simulink model "myrobot"  (R2019b)
(part 5 of 7)

-theta2_dot.*(((cos(theta1).*cos(theta2).*sin(theta3).*6.228833385e-1+cos(theta1).*cos(theta3).*sin(theta2).*6.228833385e-1).*(cos(theta1).*cos(theta2).*(4.3e+1./1.0e+2)-cos(theta1).*sin(theta2).*sin(theta3).*1.20975e-1+cos(theta1).*cos(theta2).*cos(theta3).*1.20975e-1))./2.0+((cos(theta2).*sin(theta1).*sin(theta3).*6.228833385e-1+cos(theta3).*sin(theta1).*sin(theta2).*6.228833385e-1).*(cos(theta2).*sin(theta1).*(4.3e+1./1.0e+2)-sin(theta1).*sin(theta2).*sin(theta3).*1.20975e-1+cos(theta2).*cos(theta3).*sin(theta1).*1.20975e-1))./2.0-((cos(theta2).*cos(theta3).*1.20975e-1-sin(theta2).*sin(theta3).*1.20975e-1).*(sin(theta2).*2.2140098+cos(theta2).*sin(theta3).*6.228833385e-1+cos(theta3).*sin(theta2).*6.228833385e-1))./2.0+((cos(theta1).*cos(theta2).*sin(theta3).*1.20975e-1+cos(theta1).*cos(theta3).*sin(theta2).*1.20975e-1).*(cos(theta1).*cos(theta2).*2.2140098-cos(theta1).*sin(theta2).*sin(theta3).*6.228833385e-1+cos(theta1).*cos(theta2).*cos(theta3).*6.228833385e-1))./2.0+(cos(theta1).*(sin(theta1).*(cos(theta1).*(cos(theta1).*sin(theta2).*sin(theta3).*(-2.74946e-3)+cos(theta1).*cos(theta2).*cos(theta3).*2.74946e-3+cos(theta1).*cos(theta2).*sin(theta3).*2.13561e-9+cos(theta1).*cos(theta3).*sin(theta2).*2.13561e-9)+(cos(theta2).*sin(theta1).*sin(theta3)+cos(theta3).*sin(theta1).*sin(theta2)).*(sin(theta1).*(-2.13561e-9)+cos(theta1).*sin(theta2).*sin(theta3).*7.5434e-2-cos(theta1).*cos(theta2).*cos(theta3).*7.5434e-2+cos(theta1).*cos(theta2).*sin(theta3).*2.67415e-8+cos(theta1).*cos(theta3).*sin(theta2).*2.67415e-8)+(cos(theta2).*sin(theta1).*sin(theta3)+cos(theta3).*sin(theta1).*sin(theta2)).*(cos(theta1).*sin(theta2).*sin(theta3).*(-1.0425e-2)+cos(theta1).*cos(theta2).*cos(theta3).*1.0425e-2+cos(theta1).*cos(theta2).*sin(theta3).*2.67415e-8+cos(theta1).*cos(theta3).*sin(theta2).*2.67415e-8)+(sin(theta1).*sin(theta2).*sin(theta3)-cos(theta2).*cos(theta3).*sin(theta1)).*(cos(theta1).*sin(theta2).*sin(theta3).*(-2.67415e-8)+cos(theta1).*cos(theta2).*cos(theta3).*2.67415e-8+cos(theta1).*cos(theta2).*sin(theta3).*7.5434e-2+cos(theta1).*cos(theta3).*sin(theta2).*7.5434e-2)-(sin(theta1).*sin(theta2).*sin(theta3)-cos(theta2).*cos(theta3).*sin(theta1)).*(sin(theta1).*(-2.74946e-3)+cos(theta1).*sin(theta2).*sin(theta3).*2.67415e-8-cos(theta1).*cos(theta2).*cos(theta3).*2.67415e-8+cos(theta1).*cos(theta2).*sin(theta3).*1.0425e-2+cos(theta1).*cos(theta3).*sin(theta2).*1.0425e-2))-cos(theta1).*((sin(theta1).*sin(theta2).*sin(theta3)-cos(theta2).*cos(theta3).*sin(theta1)).*(cos(theta2).*sin(theta1).*sin(theta3).*7.5434e-2+cos(theta3).*sin(theta1).*sin(theta2).*7.5434e-2-sin(theta1).*sin(theta2).*sin(theta3).*2.67415e-8+cos(theta2).*cos(theta3).*sin(theta1).*2.67415e-8)-(sin(theta1).*sin(theta2).*sin(theta3)-cos(theta2).*cos(theta3).*sin(theta1)).*(cos(theta1).*2.74946e-3+cos(theta2).*sin(theta1).*sin(theta3).*1.0425e-2+cos(theta3).*sin(theta1).*sin(theta2).*1.0425e-2+sin(theta1).*sin(theta2).*sin(theta3).*2.67415e-8-cos(theta2).*cos(theta3).*sin(theta1).*2.67415e-8)+(cos(theta2).*sin(theta1).*sin(theta3)+cos(theta3).*sin(theta1).*sin(theta2)).*(cos(theta1).*2.13561e-9+cos(theta2).*sin(theta1).*sin(theta3).*2.67415e-8+cos(theta3).*sin(theta1).*sin(theta2).*2.67415e-8+sin(theta1).*sin(theta2).*sin(theta3).*7.5434e-2-cos(theta2).*cos(theta3).*sin(theta1).*7.5434e-2)+cos(theta1).*(cos(theta2).*sin(theta1).*sin(theta3).*2.13561e-9+cos(theta3).*sin(theta1).*sin(theta2).*2.13561e-9-sin(theta1).*sin(theta2).*sin(theta3).*2.74946e-3+cos(theta2).*cos(theta3).*sin(theta1).*2.74946e-3)+(cos(theta2).*sin(theta1).*sin(theta3)+cos(theta3).*sin(theta1).*sin(theta2)).*(cos(theta2).*sin(theta1).*sin(theta3).*2.67415e-8+cos(theta3).*sin(theta1).*sin(theta2).*2.67415e-8-sin(theta1).*sin(theta2).*sin(theta3).*1.0425e-2+cos(theta2).*cos(theta3).*sin(theta1).*1.0425e-2))))./2.0+((cos(theta2).*sin(theta1).*sin(theta3).*1.20975e-1+cos(theta3).*sin(theta1).*sin(theta2).*1.20975e-1).*(cos(theta2).*sin(theta1).*2.2140098-sin(theta1).*sin(theta2).*sin(theta3).*6.228833385e-1+cos(theta2).*cos(theta3).*sin(theta1).*6.228833385e-1))./2.0-((cos(theta2).*cos(theta3).*6.228833385e-1-sin(theta2).*sin(theta3).*6.228833385e-1).*(sin(theta2).*(4.3e+1./1.0e+2)+cos(theta2).*sin(theta3).*1.20975e-1+cos(theta3).*sin(theta2).*1.20975e-1))./2.0-(sin(theta1).*(sin(theta1).*((cos(theta1).*cos(theta2).*sin(theta3)+cos(theta1).*cos(theta3).*sin(theta2)).*(sin(theta1).*(-2.13561e-9)+cos(theta1).*sin(theta2).*sin(theta3).*7.5434e-2-cos(theta1).*cos(theta2).*cos(theta3).*7.5434e-2+cos(theta1).*cos(theta2).*sin(theta3).*2.67415e-8+cos(theta1).*cos(theta3).*sin(theta2).*2.67415e-8)+(cos(theta1).*cos(theta2).*sin(theta3)+cos(theta1).*cos(theta3).*sin(theta2)).*(cos(theta1).*sin(theta2).*sin(theta3).*(-1.0425e-2)+cos(theta1).*cos(theta2).*cos(theta3).*1.0425e-2+cos(theta1).*cos(theta2).*sin(theta3).*2.67415e-8+cos(theta1).*cos(theta3).*sin(theta2).*2.67415e-8)-sin(theta1).*(cos(theta1).*sin(theta2).*sin(theta3).*(-2.74946e-3)+cos(theta1).*cos(theta2).*cos(theta3).*2.74946e-3+cos(theta1).*cos(theta2).*sin(theta3).*2.13561e-9+cos(theta1).*cos(theta3).*sin(theta2).*2.13561e-9)+(cos(theta1).*sin(theta2).*sin(theta3)-cos(theta1).*cos(theta2).*cos(theta3)).*(cos(theta1).*sin(theta2).*sin(theta3).*(-2.67415e-8)+cos(theta1).*cos(theta2).*cos(theta3).*2.67415e-8+cos(theta1).*cos(theta2).*sin(theta3).*7.5434e-2+cos(theta1).*cos(theta3).*sin(theta2).*7.5434e-2)-(cos(theta1).*sin(theta2).*sin(theta3)-cos(theta1).*cos(theta2).*cos(theta3)).*(sin(theta1).*(-2.74946e-3)+cos(theta1).*sin(theta2).*sin(theta3).*2.67415e-8-cos(theta1).*cos(theta2).*cos(theta3).*2.67415e-8+cos(theta1).*cos(theta2).*sin(theta3).*1.0425e-2+cos(theta1).*cos(theta3).*sin(theta2).*1.0425e-2))-cos(theta1).*((cos(theta1).*cos(theta2).*sin(theta3)+cos(theta1).*cos(theta3).*sin(theta2)).*(cos(theta1).*2.13561e-9+cos(theta2).*sin(theta1).*sin(theta3).*2.67415e-8+cos(theta3).*sin(theta1).*sin(theta2).*2.67415e-8+sin(theta1).*sin(theta2).*sin(theta3).*7.5434e-2-cos(theta2).*cos(theta3).*sin(theta1).*7.5434e-2)+(cos(theta1).*cos(theta2).*sin(theta3)+cos(theta1).*cos(theta3).*sin(theta2)).*(cos(theta2).*sin(theta1).*sin(theta3).*2.67415e-8+cos(theta3).*sin(theta1).*sin(theta2).*2.67415e-8-sin(theta1).*sin(theta2).*sin(theta3).*1.0425e-2+cos(theta2).*cos(theta3).*sin(theta1).*1.0425e-2)-sin(theta1).*(cos(theta2).*sin(theta1).*sin(theta3).*2.13561e-9+cos(theta3).*sin(theta1).*sin(theta2).*2.13561e-9-sin(theta1).*sin(theta2).*sin(theta3).*2.74946e-3+cos(theta2).*cos(theta3).*sin(theta1).*2.74946e-3)+(cos(theta1).*sin(theta2).*sin(theta3)-cos(theta1).*cos(theta2).*cos(theta3)).*(cos(theta2).*sin(theta1).*sin(theta3).*7.5434e-2+cos(theta3).*sin(theta1).*sin(theta2).*7.5434e-2-sin(theta1).*sin(theta2).*sin(theta3).*2.67415e-8+cos(theta2).*cos(theta3).*sin(theta1).*2.67415e-8)-(cos(theta1).*sin(theta2).*sin(theta3)-cos(theta1).*cos(theta2).*cos(theta3)).*(cos(theta1).*2.74946e-3+cos(theta2).*sin(theta1).*sin(theta3).*1.0425e-2+cos(theta3).*sin(theta1).*sin(theta2).*1.0425e-2+sin(theta1).*sin(theta2).*sin(theta3).*2.67415e-8-cos(theta2).*cos(theta3).*sin(theta1).*2.67415e-8))))./2.0)-theta3_dot.*(((cos(theta2).*sin(theta1).*sin(theta3).*1.20975e-1+cos(theta3).*sin(theta1).*sin(theta2).*1.20975e-1).*(sin(theta1).*sin(theta2).*sin(theta3).*6.228833385e-1-cos(theta2).*cos(theta3).*sin(theta1).*6.228833385e-1))./2.0-((sin(theta1).*sin(theta2).*sin(theta3).*1.20975e-1-cos(theta2).*cos(theta3).*sin(theta1).*1.20975e-1).*(cos(theta2).*sin(theta1).*sin(theta3).*6.228833385e-1+cos(theta3).*sin(theta1).*sin(theta2).*6.228833385e-1))./2.0-(cos(theta2).*cos(theta3).*1.20975e-1-sin(theta2).*sin(theta3).*1.20975e-1).*(sin(theta2).*2.2140098+cos(theta2).*sin(theta3).*6.228833385e-1+cos(theta3).*sin(theta2).*6.228833385e-1)+(cos(theta1).*cos(theta2).*sin(theta3).*1.20975e-1+cos(theta1).*cos(theta3).*sin(theta2).*1.20975e-1).*(cos(theta1).*cos(theta2).*2.2140098-cos(theta1).*sin(theta2).*sin(theta3).*6.228833385e-1+cos(theta1).*cos(theta2).*cos(theta3).*6.228833385e-1)+((cos(theta2).*cos(theta3).*1.20975e-1-sin(theta2).*sin(theta3).*1.20975e-1).*(cos(theta2).*sin(theta3).*6.228833385e-1+cos(theta3).*sin(theta2).*6.228833385e-1))./2.0-((cos(theta2).*sin(theta3).*1.20975e-1+cos(theta3).*sin(theta2).*1.20975e-1).*(cos(theta2).*cos(theta3).*6.228833385e-1-sin(theta2).*sin(theta3).*6.228833385e-1))./2.0+(cos(theta1).*(sin(theta1).*(cos(theta1).*(cos(theta1).*sin(theta2).*sin(theta3).*(-2.74946e-3)+cos(theta1).*cos(theta2).*cos(theta3).*2.74946e-3+cos(theta1).*cos(theta2).*sin(theta3).*2.13561e-9+cos(theta1).*cos(theta3).*sin(theta2).*2.13561e-9)+(cos(theta2).*sin(theta1).*sin(theta3)+cos(theta3).*sin(theta1).*sin(theta2)).*(sin(theta1).*(-2.13561e-9)+cos(theta1).*sin(theta2).*sin(theta3).*7.5434e-2-cos(theta1).*cos(theta2).*cos(theta3).*7.5434e-2+cos(theta1).*cos(theta2).*sin(theta3).*2.67415e-8+cos(theta1).*cos(theta3).*sin(theta2).*2.67415e-8)+(cos(theta2).*sin(theta1).*sin(theta3)+cos(theta3).*sin(theta1).*sin(theta2)).*(cos(theta1).*sin(theta2).*sin(theta3).*(-1.0425e-2)+cos(theta1).*cos(theta2).*cos(theta3).*1.0425e-2+cos(theta1).*cos(theta2).*sin(theta3).*2.67415e-8+cos(theta1).*cos(theta3).*sin(theta2).*2.67415e-8)+(sin(theta1).*sin(theta2).*sin(theta3)-cos(theta2).*cos(theta3).*sin(theta1)).*(cos(theta1).*sin(theta2).*sin(theta3).*(-2.67415e-8)+cos(theta1).*cos(theta2).*cos(theta3).*2.67415e-8+cos(theta1).*cos(theta2).*sin(theta3).*7.5434e-2+cos(theta1).*cos(theta3).*sin(theta2).*7.5434e-2)-(sin(theta1).*sin(theta2).*sin(theta3)-cos(theta2).*cos(theta3).*sin(theta1)).*(sin(theta1).*(-2.74946e-3)+cos(theta1).*sin(theta2).*sin(theta3).*2.67415e-8-cos(theta1).*cos(theta2).*cos(theta3).*2.67415e-8+cos(theta1).*cos(theta2).*sin(theta3).*1.0425e-2+cos(theta1).*cos(theta3).*sin(theta2).*1.0425e-2))-cos(theta1).*((sin(theta1).*sin(theta2).*sin(theta3)-cos(theta2).*cos(theta3).*sin(theta1)).*(cos(theta2).*sin(theta1).*sin(theta3).*7.5434e-2+cos(theta3).*sin(theta1).*sin(theta2).*7.5434e-2-sin(theta1).*sin(theta2).*sin(theta3).*2.67415e-8+cos(theta2).*cos(theta3).*sin(theta1).*2.67415e-8)-(sin(theta1).*sin(theta2).*sin(theta3)-cos(theta2).*cos(theta3).*sin(theta1)).*(cos(theta1).*2.74946e-3+cos(theta2).*sin(theta1).*sin(theta3).*1.0425e-2+cos(theta3).*sin(theta1).*sin(theta2).*1.0425e-2+sin(theta1).*sin(theta2).*sin(theta3).*2.67415e-8-cos(theta2).*cos(theta3).*sin(theta1).*2.67415e-8)+(cos(theta2).*sin(theta1).*sin(theta3)+cos(theta3).*sin(theta1).*sin(theta2)).*(cos(theta1).*2.13561e-9+cos(theta2).*sin(theta1).*sin(theta3).*2.67415e-8+cos(theta3).*sin(theta1).*sin(theta2).*2.67415e-8+sin(theta1).*sin(theta2).*sin(theta3).*7.5434e-2-cos(theta2).*cos(theta3).*sin(theta1).*7.5434e-2)+cos(theta1).*(cos(theta2).*sin(theta1).*sin(theta3).*2.13561e-9+cos(theta3).*sin(theta1).*sin(theta2).*2.13561e-9-sin(theta1).*sin(theta2).*sin(theta3).*2.74946e-3+cos(theta2).*cos(theta3).*sin(theta1).*2.74946e-3)+(cos(theta2).*sin(theta1).*sin(theta3)+cos(theta3).*sin(theta1).*sin(theta2)).*(cos(theta2).*sin(theta1).*sin(theta3).*2.67415e-8+cos(theta3).*sin(theta1).*sin(theta2).*2.67415e-8-sin(theta1).*sin(theta2).*sin(theta3).*1.0425e-2+cos(theta2).*cos(theta3).*sin(theta1).*1.0425e-2))))./2.0+(cos(theta2).*sin(theta1).*sin(theta3).*1.20975e-1+cos(theta3).*sin(theta1).*sin(theta2).*1.20975e-1).*(cos(theta2).*sin(theta1).*2.2140098-sin(theta1).*sin(theta2).*sin(theta3).*6.228833385e-1+cos(theta2).*cos(theta3).*sin(theta1).*6.228833385e-1)-(sin(theta1).*(sin(theta1).*((cos(theta1).*cos(theta2).*sin(theta3)+cos(theta1).*cos(theta3).*sin(theta2)).*(sin(theta1).*(-2.13561e-9)+cos(theta1).*sin(theta2).*sin(theta3).*7.5434e-2-cos(theta1).*cos(theta2).*cos(theta3).*7.5434e-2+cos(theta1).*cos(theta2).*sin(theta3).*2.67415e-8+cos(theta1).*cos(theta3).*sin(theta2).*2.67415e-8)+(cos(theta1).*cos(theta2).*sin(theta3)+cos(theta1).*cos(theta3).*sin(theta2)).*(cos(theta1).*sin(theta2).*sin(theta3).*(-1.0425e-2)+cos(theta1).*cos(theta2).*cos(theta3).*1.0425e-2+cos(theta1).*cos(theta2).*sin(theta3).*2.67415e-8+cos(theta1).*cos(theta3).*sin(theta2).*2.67415e-8)-sin(theta1).*(cos(theta1).*sin(theta2).*sin(theta3).*(-2.74946e-3)+cos(theta1).*cos(theta2).*cos(theta3).*2.74946e-3+cos(theta1).*cos(theta2).*sin(theta3).*2.13561e-9+cos(theta1).*cos(theta3).*sin(theta2).*2.13561e-9)+(cos(theta1).*sin(theta2).*sin(theta3)-cos(theta1).*cos(theta2).*cos(theta3)).*(cos(theta1).*sin(theta2).*sin(theta3).*(-2.67415e-8)+cos(theta1).*cos(theta2).*cos(theta3).*2.67415e-8+cos(theta1).*cos(theta2).*sin(theta3).*7.5434e-2+cos(theta1).*cos(theta3).*sin(theta2).*7.5434e-2)-(cos(theta1).*sin(theta2).*sin(theta3)-cos(theta1).*cos(theta2).*cos(theta3)).*(sin(theta1).*(-2.74946e-3)+cos(theta1).*sin(theta2).*sin(theta3).*2.67415e-8-cos(theta1).*cos(theta2).*cos(theta3).*2.67415e-8+cos(theta1).*cos(theta2).*sin(theta3).*1.0425e-2+cos(theta1).*cos(theta3).*sin(theta2).*1.0425e-2))-cos(theta1).*((cos(theta1).*cos(theta2).*sin(theta3)+cos(theta1).*cos(theta3).*sin(theta2)).*(cos(theta1).*2.13561e-9+cos(theta2).*sin(theta1).*sin(theta3).*2.67415e-8+cos(theta3).*sin(theta1).*sin(theta2).*2.67415e-8+sin(theta1).*sin(theta2).*sin(theta3).*7.5434e-2-cos(theta2).*cos(theta3).*sin(theta1).*7.5434e-2)+(cos(theta1).*cos(theta2).*sin(theta3)+cos(theta1).*cos(theta3).*sin(theta2)).*(cos(theta2).*sin(theta1).*sin(theta3).*2.67415e-8+cos(theta3).*sin(theta1).*sin(theta2).*2.67415e-8-sin(theta1).*sin(theta2).*sin(theta3).*1.0425e-2+cos(theta2).*cos(theta3).*sin(theta1).*1.0425e-2)-sin(theta1).*(cos(theta2).*sin(theta1).*sin(theta3).*2.13561e-9+cos(theta3).*sin(theta1).*sin(theta2).*2.13561e-9-sin(theta1).*sin(theta2).*sin(theta3).*2.74946e-3+cos(theta2).*cos(theta3).*sin(theta1).*2.74946e-3)+(cos(theta1).*sin(theta2).*sin(theta3)-cos(theta1).*cos(theta2).*cos(theta3)).*(cos(theta2).*sin(theta1).*sin(theta3).*7.5434e-2+cos(theta3).*sin(theta1).*sin(theta2).*7.5434e-2-sin(theta1).*sin(theta2).*sin(theta3).*2.67415e-8+cos(theta2).*cos(theta3).*sin(theta1).*2.67415e-8)-(cos(theta1).*sin(theta2).*sin(theta3)-cos(theta1).*cos(theta2).*cos(theta3)).*(cos(theta1).*2.74946e-3+cos(theta2).*sin(theta1).*sin(theta3).*1.0425e-2+cos(theta3).*sin(theta1).*sin(theta2).*1.0425e-2+sin(theta1).*sin(theta2).*sin(theta3).*2.67415e-8-cos(theta2).*cos(theta3).*sin(theta1).*2.67415e-8))))./2.0-((cos(theta1).*sin(theta2).*sin(theta3).*1.20975e-1-cos(theta1).*cos(theta2).*cos(theta3).*1.20975e-1).*(cos(theta1).*cos(theta2).*sin(theta3).*6.228833385e-1+cos(theta1).*cos(theta3).*sin(theta2).*6.228833385e-1))./2.0+((cos(theta1).*cos(theta2).*sin(theta3).*1.20975e-1+cos(theta1).*cos(theta3).*sin(theta2).*1.20975e-1).*(cos(theta1).*sin(theta2).*sin(theta3).*6.228833385e-1-cos(theta1).*cos(theta2).*cos(theta3).*6.228833385e-1))./2.0)-theta1_dot.*((cos(theta1).*(cos(theta1).*(cos(theta1).*(sin(theta1).*(-7.44749e-2)+cos(theta1).*sin(theta2).*sin(theta3).*2.13561e-9-cos(theta1).*cos(theta2).*cos(theta3).*2.13561e-9+cos(theta1).*cos(theta2).*sin(theta3).*2.74946e-3+cos(theta1).*cos(theta3).*sin(theta2).*2.74946e-3)+(sin(theta1).*sin(theta2).*sin(theta3)-cos(theta2).*cos(theta3).*sin(theta1)).*(sin(theta1).*(-2.13561e-9)+cos(theta1).*sin(theta2).*sin(theta3).*7.5434e-2-cos(theta1).*cos(theta2).*cos(theta3).*7.5434e-2+cos(theta1).*cos(theta2).*sin(theta3).*2.67415e-8+cos(theta1).*cos(theta3).*sin(theta2).*2.67415e-8)+(cos(theta2).*sin(theta1).*sin(theta3)+cos(theta3).*sin(theta1).*sin(theta2)).*(sin(theta1).*(-2.74946e-3)+cos(theta1).*sin(theta2).*sin(theta3).*2.67415e-8-cos(theta1).*cos(theta2).*cos(theta3).*2.67415e-8+cos(theta1).*cos(theta2).*sin(theta3).*1.0425e-2+cos(theta1).*cos(theta3).*sin(theta2).*1.0425e-2))+sin(theta1).*((cos(theta2).*sin(theta1).*sin(theta3)+cos(theta3).*sin(theta1).*sin(theta2)).*(cos(theta1).*2.74946e-3+cos(theta2).*sin(theta1).*sin(theta3).*1.0425e-2+cos(theta3).*sin(theta1).*sin(theta2).*1.0425e-2+sin(theta1).*sin(theta2).*sin(theta3).*2.67415e-8-cos(theta2).*cos(theta3).*sin(theta1).*2.67415e-8)+cos(theta1).*(cos(theta1).*7.44749e-2+cos(theta2).*sin(theta1).*sin(theta3).*2.74946e-3+cos(theta3).*sin(theta1).*sin(theta2).*2.74946e-3+sin(theta1).*sin(theta2).*sin(theta3).*2.13561e-9-cos(theta2).*cos(theta3).*sin(theta1).*2.13561e-9)+(sin(theta1).*sin(theta2).*sin(theta3)-cos(theta2).*cos(theta3).*sin(theta1)).*(cos(theta1).*2.13561e-9+cos(theta2).*sin(theta1).*sin(theta3).*2.67415e-8+cos(theta3).*sin(theta1).*sin(theta2).*2.67415e-8+sin(theta1).*sin(theta2).*sin(theta3).*7.5434e-2-cos(theta2).*cos(theta3).*sin(theta1).*7.5434e-2))-cos(theta1).*(cos(theta1).*(sin(theta1).*(-7.44749e-2)+cos(theta1).*sin(theta2).*sin(theta3).*2.13561e-9-cos(theta1).*cos(theta2).*cos(theta3).*2.13561e-9+cos(theta1).*cos(theta2).*sin(theta3).*2.74946e-3+cos(theta1).*cos(theta3).*sin(theta2).*2.74946e-3)+(sin(theta1).*sin(theta2).*sin(theta3)-cos(theta2).*cos(theta3).*sin(theta1)).*(sin(theta1).*(-2.13561e-9)+cos(theta1).*sin(theta2).*sin(theta3).*7.5434e-2-cos(theta1).*cos(theta2).*cos(theta3).*7.5434e-2+cos(theta1).*cos(theta2).*sin(theta3).*2.67415e-8+cos(theta1).*cos(theta3).*sin(theta2).*2.67415e-8)-sin(theta1).*(cos(theta1).*7.44749e-2+cos(theta2).*sin(theta1).*sin(theta3).*2.74946e-3+cos(theta3).*sin(theta1).*sin(theta2).*2.74946e-3+sin(theta1).*sin(theta2).*sin(theta3).*2.13561e-9-cos(theta2).*cos(theta3).*sin(theta1).*2.13561e-9)+(cos(theta1).*sin(theta2).*sin(theta3)-cos(theta1).*cos(theta2).*cos(theta3)).*(cos(theta1).*2.13561e-9+cos(theta2).*sin(theta1).*sin(theta3).*2.67415e-8+cos(theta3).*sin(theta1).*sin(theta2).*2.67415e-8+sin(theta1).*sin(theta2).*sin(theta3).*7.5434e-2-cos(theta2).*cos(theta3).*sin(theta1).*7.5434e-2)+(cos(theta2).*sin(theta1).*sin(theta3)+cos(theta3).*sin(theta1).*sin(theta2)).*(sin(theta1).*(-2.74946e-3)+cos(theta1).*sin(theta2).*sin(theta3).*2.67415e-8-cos(theta1).*cos(theta2).*cos(theta3).*2.67415e-8+cos(theta1).*cos(theta2).*sin(theta3).*1.0425e-2+cos(theta1).*cos(theta3).*sin(theta2).*1.0425e-2)+(cos(theta1).*cos(theta2).*sin(theta3)+cos(theta1).*cos(theta3).*sin(theta2)).*(cos(theta1).*2.74946e-3+cos(theta2).*sin(theta1).*sin(theta3).*1.0425e-2+cos(theta3).*sin(theta1).*sin(theta2).*1.0425e-2+sin(theta1).*sin(theta2).*sin(theta3).*2.67415e-8-cos(theta2).*cos(theta3).*sin(theta1).*2.67415e-8))-sin(theta1).*((cos(theta2).*sin(theta1).*sin(theta3)+cos(theta3).*sin(theta1).*sin(theta2)).*(cos(theta1).*2.74946e-3+cos(theta2).*sin(theta1).*sin(theta3).*1.0425e-2+cos(theta3).*sin(theta1).*sin(theta2).*1.0425e-2+sin(theta1).*sin(theta2).*sin(theta3).*2.67415e-8-cos(theta2).*cos(theta3).*sin(theta1).*2.67415e-8)+sin(theta1).*(sin(theta1).*(-7.44749e-2)+cos(theta1).*sin(theta2).*sin(theta3).*2.13561e-9-cos(theta1).*cos(theta2).*cos(theta3).*2.13561e-9+cos(theta1).*cos(theta2).*sin(theta3).*2.74946e-3+cos(theta1).*cos(theta3).*sin(theta2).*2.74946e-3)-(cos(theta1).*sin(theta2).*sin(theta3)-cos(theta1).*cos(theta2).*cos(theta3)).*(sin(theta1).*(-2.13561e-9)+cos(theta1).*sin(theta2).*sin(theta3).*7.5434e-2-cos(theta1).*cos(theta2).*cos(theta3).*7.5434e-2+cos(theta1).*cos(theta2).*sin(theta3).*2.67415e-8+cos(theta1).*cos(theta3).*sin(theta2).*2.67415e-8)+cos(theta1).*(cos(theta1).*7.44749e-2+cos(theta2).*sin(theta1).*sin(theta3).*2.74946e-3+cos(theta3).*sin(theta1).*sin(theta2).*2.74946e-3+sin(theta1).*sin(theta2).*sin(theta3).*2.13561e-9-cos(theta2).*cos(theta3).*sin(theta1).*2.13561e-9)+(sin(theta1).*sin(theta2).*sin(theta3)-cos(theta2).*cos(theta3).*sin(theta1)).*(cos(theta1).*2.13561e-9+cos(theta2).*sin(theta1).*sin(theta3).*2.67415e-8+cos(theta3).*sin(theta1).*sin(theta2).*2.67415e-8+sin(theta1).*sin(theta2).*sin(theta3).*7.5434e-2-cos(theta2).*cos(theta3).*sin(theta1).*7.5434e-2)-(cos(theta1).*cos(theta2).*sin(theta3)+cos(theta1).*cos(theta3).*sin(theta2)).*(sin(theta1).*(-2.74946e-3)+cos(theta1).*sin(theta2).*sin(theta3).*2.67415e-8-cos(theta1).*cos(theta2).*cos(theta3).*2.67415e-8+cos(theta1).*cos(theta2).*sin(theta3).*1.0425e-2+cos(theta1).*cos(theta3).*sin(theta2).*1.0425e-2))))./2.0+((cos(theta1).*cos(theta2).*sin(theta3).*1.20975e-1+cos(theta1).*cos(theta3).*sin(theta2).*1.20975e-1).*(cos(theta1).*2.272809781200003e-2+sin(theta1).*sin(theta2).*2.2140098+cos(theta2).*sin(theta1).*sin(theta3).*6.228833385e-1+cos(theta3).*sin(theta1).*sin(theta2).*6.228833385e-1))./2.0-((cos(theta2).*sin(theta1).*sin(theta3).*1.20975e-1+cos(theta3).*sin(theta1).*sin(theta2).*1.20975e-1).*(sin(theta1).*(-2.272809781200003e-2)+cos(theta1).*sin(theta2).*2.2140098+cos(theta1).*cos(theta2).*sin(theta3).*6.228833385e-1+cos(theta1).*cos(theta3).*sin(theta2).*6.228833385e-1))./2.0-((cos(theta1).*cos(theta2).*sin(theta3).*6.228833385e-1+cos(theta1).*cos(theta3).*sin(theta2).*6.228833385e-1).*(cos(theta1).*4.414200000000005e-3+sin(theta1).*sin(theta2).*(4.3e+1./1.0e+2)+cos(theta2).*sin(theta1).*sin(theta3).*1.20975e-1+cos(theta3).*sin(theta1).*sin(theta2).*1.20975e-1))./2.0+((cos(theta2).*sin(theta1).*sin(theta3).*6.228833385e-1+cos(theta3).*sin(theta1).*sin(theta2).*6.228833385e-1).*(sin(theta1).*(-4.414200000000005e-3)+cos(theta1).*sin(theta2).*(4.3e+1./1.0e+2)+cos(theta1).*cos(theta2).*sin(theta3).*1.20975e-1+cos(theta1).*cos(theta3).*sin(theta2).*1.20975e-1))./2.0+(sin(theta1).*(-sin(theta1).*(cos(theta2).*cos(theta3).*(-2.13561e-9)+cos(theta2).*sin(theta3).*2.74946e-3+cos(theta3).*sin(theta2).*2.74946e-3+sin(theta2).*sin(theta3).*2.13561e-9)-(cos(theta1).*cos(theta2).*sin(theta3)+cos(theta1).*cos(theta3).*sin(theta2)).*(cos(theta2).*cos(theta3).*2.67415e-8+cos(theta2).*sin(theta3).*7.5434e-2+cos(theta3).*sin(theta2).*7.5434e-2-sin(theta2).*sin(theta3).*2.67415e-8)+(cos(theta1).*sin(theta2).*sin(theta3)-cos(theta1).*cos(theta2).*cos(theta3)).*(cos(theta2).*cos(theta3).*(-7.5434e-2)+cos(theta2).*sin(theta3).*2.67415e-8+cos(theta3).*sin(theta2).*2.67415e-8+sin(theta2).*sin(theta3).*7.5434e-2)+(cos(theta1).*cos(theta2).*sin(theta3)+cos(theta1).*cos(theta3).*sin(theta2)).*(cos(theta2).*cos(theta3).*(-2.67415e-8)+cos(theta2).*sin(theta3).*1.0425e-2+cos(theta3).*sin(theta2).*1.0425e-2+sin(theta2).*sin(theta3).*2.67415e-8)+(cos(theta1).*sin(theta2).*sin(theta3)-cos(theta1).*cos(theta2).*cos(theta3)).*(cos(theta2).*cos(theta3).*1.0425e-2+cos(theta2).*sin(theta3).*2.67415e-8+cos(theta3).*sin(theta2).*2.67415e-8-sin(theta2).*sin(theta3).*1.0425e-2)))./2.0-(sin(theta1).*(sin(theta1).*(cos(theta1).*(sin(theta1).*(-7.44749e-2)+cos(theta1).*sin(theta2).*sin(theta3).*2.13561e-9-cos(theta1).*cos(theta2).*cos(theta3).*2.13561e-9+cos(theta1).*cos(theta2).*sin(theta3).*2.74946e-3+cos(theta1).*cos(theta3).*sin(theta2).*2.74946e-3)+(sin(theta1).*sin(theta2).*sin(theta3)-cos(theta2).*cos(theta3).*sin(theta1)).*(sin(theta1).*(-2.13561e-9)+cos(theta1).*sin(theta2).*sin(theta3).*7.5434e-2-cos(theta1).*cos(theta2).*cos(theta3).*7.5434e-2+cos(theta1).*cos(theta2).*sin(theta3).*2.67415e-8+cos(theta1).*cos(theta3).*sin(theta2).*2.67415e-8)+(cos(theta2).*sin(theta1).*sin(theta3)+cos(theta3).*sin(theta1).*sin(theta2)).*(sin(theta1).*(-2.74946e-3)+cos(theta1).*sin(theta2).*sin(theta3).*2.67415e-8-cos(theta1).*cos(theta2).*cos(theta3).*2.67415e-8+cos(theta1).*cos(theta2).*sin(theta3).*1.0425e-2+cos(theta1).*cos(theta3).*sin(theta2).*1.0425e-2))-cos(theta1).*((cos(theta2).*sin(theta1).*sin(theta3)+cos(theta3).*sin(theta1).*sin(theta2)).*(cos(theta1).*2.74946e-3+cos(theta2).*sin(theta1).*sin(theta3).*1.0425e-2+cos(theta3).*sin(theta1).*sin(theta2).*1.0425e-2+sin(theta1).*sin(theta2).*sin(theta3).*2.67415e-8-cos(theta2).*cos(theta3).*sin(theta1).*2.67415e-8)+cos(theta1).*(cos(theta1).*7.44749e-2+cos(theta2).*sin(theta1).*sin(theta3).*2.74946e-3+cos(theta3).*sin(theta1).*sin(theta2).*2.74946e-3+sin(theta1).*sin(theta2).*sin(theta3).*2.13561e-9-cos(theta2).*cos(theta3).*sin(theta1).*2.13561e-9)+(sin(theta1).*sin(theta2).*sin(theta3)-cos(theta2).*cos(theta3).*sin(theta1)).*(cos(theta1).*2.13561e-9+cos(theta2).*sin(theta1).*sin(theta3).*2.67415e-8+cos(theta3).*sin(theta1).*sin(theta2).*2.67415e-8+sin(theta1).*sin(theta2).*sin(theta3).*7.5434e-2-cos(theta2).*cos(theta3).*sin(theta1).*7.5434e-2))))./2.0-(cos(theta1).*(cos(theta1).*(cos(theta2).*cos(theta3).*(-2.13561e-9)+cos(theta2).*sin(theta3).*2.74946e-3+cos(theta3).*sin(theta2).*2.74946e-3+sin(theta2).*sin(theta3).*2.13561e-9)+(cos(theta2).*sin(theta1).*sin(theta3)+cos(theta3).*sin(theta1).*sin(theta2)).*(cos(theta2).*cos(theta3).*(-2.67415e-8)+cos(theta2).*sin(theta3).*1.0425e-2+cos(theta3).*sin(theta2).*1.0425e-2+sin(theta2).*sin(theta3).*2.67415e-8)+(sin(theta1).*sin(theta2).*sin(theta3)-cos(theta2).*cos(theta3).*sin(theta1)).*(cos(theta2).*cos(theta3).*1.0425e-2+cos(theta2).*sin(theta3).*2.67415e-8+cos(theta3).*sin(theta2).*2.67415e-8-sin(theta2).*sin(theta3).*1.0425e-2)-(cos(theta2).*sin(theta1).*sin(theta3)+cos(theta3).*sin(theta1).*sin(theta2)).*(cos(theta2).*cos(theta3).*2.67415e-8+cos(theta2).*sin(theta3).*7.5434e-2+cos(theta3).*sin(theta2).*7.5434e-2-sin(theta2).*sin(theta3).*2.67415e-8)+(sin(theta1).*sin(theta2).*sin(theta3)-cos(theta2).*cos(theta3).*sin(theta1)).*(cos(theta2).*cos(theta3).*(-7.5434e-2)+cos(theta2).*sin(theta3).*2.67415e-8+cos(theta3).*sin(theta2).*2.67415e-8+sin(theta2).*sin(theta3).*7.5434e-2)))./2.0-(sin(theta1).*sin(theta2).*sin(theta3).*1.20975e-1-cos(theta2).*cos(theta3).*sin(theta1).*1.20975e-1).*(cos(theta1).*cos(theta2).*2.2140098-cos(theta1).*sin(theta2).*sin(theta3).*6.228833385e-1+cos(theta1).*cos(theta2).*cos(theta3).*6.228833385e-1)-(cos(theta1).*((cos(theta2).*sin(theta3)+cos(theta3).*sin(theta2)).*(cos(theta2).*sin(theta1).*sin(theta3).*7.5434e-2+cos(theta3).*sin(theta1).*sin(theta2).*7.5434e-2-sin(theta1).*sin(theta2).*sin(theta3).*2.67415e-8+cos(theta2).*cos(theta3).*sin(theta1).*2.67415e-8)-(cos(theta2).*sin(theta3)+cos(theta3).*sin(theta2)).*(cos(theta1).*2.74946e-3+cos(theta2).*sin(theta1).*sin(theta3).*1.0425e-2+cos(theta3).*sin(theta1).*sin(theta2).*1.0425e-2+sin(theta1).*sin(theta2).*sin(theta3).*2.67415e-8-cos(theta2).*cos(theta3).*sin(theta1).*2.67415e-8)+(cos(theta2).*cos(theta3)-sin(theta2).*sin(theta3)).*(cos(theta1).*2.13561e-9+cos(theta2).*sin(theta1).*sin(theta3).*2.67415e-8+cos(theta3).*sin(theta1).*sin(theta2).*2.67415e-8+sin(theta1).*sin(theta2).*sin(theta3).*7.5434e-2-cos(theta2).*cos(theta3).*sin(theta1).*7.5434e-2)+(cos(theta2).*cos(theta3)-sin(theta2).*sin(theta3)).*(cos(theta2).*sin(theta1).*sin(theta3).*2.67415e-8+cos(theta3).*sin(theta1).*sin(theta2).*2.67415e-8-sin(theta1).*sin(theta2).*sin(theta3).*1.0425e-2+cos(theta2).*cos(theta3).*sin(theta1).*1.0425e-2)))./2.0+(cos(theta1).*sin(theta2).*sin(theta3).*1.20975e-1-cos(theta1).*cos(theta2).*cos(theta3).*1.20975e-1).*(cos(theta2).*sin(theta1).*2.2140098-sin(theta1).*sin(theta2).*sin(theta3).*6.228833385e-1+cos(theta2).*cos(theta3).*sin(theta1).*6.228833385e-1)-(sin(theta1).*(sin(theta1).*(-sin(theta1).*(cos(theta1).*7.44749e-2+cos(theta2).*sin(theta1).*sin(theta3).*2.74946e-3+cos(theta3).*sin(theta1).*sin(theta2).*2.74946e-3+sin(theta1).*sin(theta2).*sin(theta3).*2.13561e-9-cos(theta2).*cos(theta3).*sin(theta1).*2.13561e-9)+(cos(theta1).*sin(theta2).*sin(theta3)-cos(theta1).*cos(theta2).*cos(theta3)).*(cos(theta1).*2.13561e-9+cos(theta2).*sin(theta1).*sin(theta3).*2.67415e-8+cos(theta3).*sin(theta1).*sin(theta2).*2.67415e-8+sin(theta1).*sin(theta2).*sin(theta3).*7.5434e-2-cos(theta2).*cos(theta3).*sin(theta1).*7.5434e-2)+(cos(theta1).*cos(theta2).*sin(theta3)+cos(theta1).*cos(theta3).*sin(theta2)).*(cos(theta1).*2.74946e-3+cos(theta2).*sin(theta1).*sin(theta3).*1.0425e-2+cos(theta3).*sin(theta1).*sin(theta2).*1.0425e-2+sin(theta1).*sin(theta2).*sin(theta3).*2.67415e-8-cos(theta2).*cos(theta3).*sin(theta1).*2.67415e-8))+cos(theta1).*(-sin(theta1).*(sin(theta1).*(-7.44749e-2)+cos(theta1).*sin(theta2).*sin(theta3).*2.13561e-9-cos(theta1).*cos(theta2).*cos(theta3).*2.13561e-9+cos(theta1).*cos(theta2).*sin(theta3).*2.74946e-3+cos(theta1).*cos(theta3).*sin(theta2).*2.74946e-3)+(cos(theta1).*sin(theta2).*sin(theta3)-cos(theta1).*cos(theta2).*cos(theta3)).*(sin(theta1).*(-2.13561e-9)+cos(theta1).*sin(theta2).*sin(theta3).*7.5434e-2-cos(theta1).*cos(theta2).*cos(theta3).*7.5434e-2+cos(theta1).*cos(theta2).*sin(theta3).*2.67415e-8+cos(theta1).*cos(theta3).*sin(theta2).*2.67415e-8)+(cos(theta1).*cos(theta2).*sin(theta3)+cos(theta1).*cos(theta3).*sin(theta2)).*(sin(theta1).*(-2.74946e-3)+cos(theta1).*sin(theta2).*sin(theta3).*2.67415e-8-cos(theta1).*cos(theta2).*cos(theta3).*2.67415e-8+cos(theta1).*cos(theta2).*sin(theta3).*1.0425e-2+cos(theta1).*cos(theta3).*sin(theta2).*1.0425e-2))+cos(theta1).*((cos(theta2).*sin(theta1).*sin(theta3)+cos(theta3).*sin(theta1).*sin(theta2)).*(cos(theta1).*2.74946e-3+cos(theta2).*sin(theta1).*sin(theta3).*1.0425e-2+cos(theta3).*sin(theta1).*sin(theta2).*1.0425e-2+sin(theta1).*sin(theta2).*sin(theta3).*2.67415e-8-cos(theta2).*cos(theta3).*sin(theta1).*2.67415e-8)+sin(theta1).*(sin(theta1).*(-7.44749e-2)+cos(theta1).*sin(theta2).*sin(theta3).*2.13561e-9-cos(theta1).*cos(theta2).*cos(theta3).*2.13561e-9+cos(theta1).*cos(theta2).*sin(theta3).*2.74946e-3+cos(theta1).*cos(theta3).*sin(theta2).*2.74946e-3)-(cos(theta1).*sin(theta2).*sin(theta3)-cos(theta1).*cos(theta2).*cos(theta3)).*(sin(theta1).*(-2.13561e-9)+cos(theta1).*sin(theta2).*sin(theta3).*7.5434e-2-cos(theta1).*cos(theta2).*cos(theta3).*7.5434e-2+cos(theta1).*cos(theta2).*sin(theta3).*2.67415e-8+cos(theta1).*cos(theta3).*sin(theta2).*2.67415e-8)+cos(theta1).*(cos(theta1).*7.44749e-2+cos(theta2).*sin(theta1).*sin(theta3).*2.74946e-3+cos(theta3).*sin(theta1).*sin(theta2).*2.74946e-3+sin(theta1).*sin(theta2).*sin(theta3).*2.13561e-9-cos(theta2).*cos(theta3).*sin(theta1).*2.13561e-9)+(sin(theta1).*sin(theta2).*sin(theta3)-cos(theta2).*cos(theta3).*sin(theta1)).*(cos(theta1).*2.13561e-9+cos(theta2).*sin(theta1).*sin(theta3).*2.67415e-8+cos(theta3).*sin(theta1).*sin(theta2).*2.67415e-8+sin(theta1).*sin(theta2).*sin(theta3).*7.5434e-2-cos(theta2).*cos(theta3).*sin(theta1).*7.5434e-2)-(cos(theta1).*cos(theta2).*sin(theta3)+cos(theta1).*cos(theta3).*sin(theta2)).*(sin(theta1).*(-2.74946e-3)+cos(theta1).*sin(theta2).*sin(theta3).*2.67415e-8-cos(theta1).*cos(theta2).*cos(theta3).*2.67415e-8+cos(theta1).*cos(theta2).*sin(theta3).*1.0425e-2+cos(theta1).*cos(theta3).*sin(theta2).*1.0425e-2))-sin(theta1).*(cos(theta1).*(sin(theta1).*(-7.44749e-2)+cos(theta1).*sin(theta2).*sin(theta3).*2.13561e-9-cos(theta1).*cos(theta2).*cos(theta3).*2.13561e-9+cos(theta1).*cos(theta2).*sin(theta3).*2.74946e-3+cos(theta1).*cos(theta3).*sin(theta2).*2.74946e-3)+(sin(theta1).*sin(theta2).*sin(theta3)-cos(theta2).*cos(theta3).*sin(theta1)).*(sin(theta1).*(-2.13561e-9)+cos(theta1).*sin(theta2).*sin(theta3).*7.5434e-2-cos(theta1).*cos(theta2).*cos(theta3).*7.5434e-2+cos(theta1).*cos(theta2).*sin(theta3).*2.67415e-8+cos(theta1).*cos(theta3).*sin(theta2).*2.67415e-8)-sin(theta1).*(cos(theta1).*7.44749e-2+cos(theta2).*sin(theta1).*sin(theta3).*2.74946e-3+cos(theta3).*sin(theta1).*sin(theta2).*2.74946e-3+sin(theta1).*sin(theta2).*sin(theta3).*2.13561e-9-cos(theta2).*cos(theta3).*sin(theta1).*2.13561e-9)+(cos(theta1).*sin(theta2).*sin(theta3)-cos(theta1).*cos(theta2).*cos(theta3)).*(cos(theta1).*2.13561e-9+cos(theta2).*sin(theta1).*sin(theta3).*2.67415e-8+cos(theta3).*sin(theta1).*sin(theta2).*2.67415e-8+sin(theta1).*sin(theta2).*sin(theta3).*7.5434e-2-cos(theta2).*cos(theta3).*sin(theta1).*7.5434e-2)+(cos(theta2).*sin(theta1).*sin(theta3)+cos(theta3).*sin(theta1).*sin(theta2)).*(sin(theta1).*(-2.74946e-3)+cos(theta1).*sin(theta2).*sin(theta3).*2.67415e-8-cos(theta1).*cos(theta2).*cos(theta3).*2.67415e-8+cos(theta1).*cos(theta2).*sin(theta3).*1.0425e-2+cos(theta1).*cos(theta3).*sin(theta2).*1.0425e-2)+(cos(theta1).*cos(theta2).*sin(theta3)+cos(theta1).*cos(theta3).*sin(theta2)).*(cos(theta1).*2.74946e-3+cos(theta2).*sin(theta1).*sin(theta3).*1.0425e-2+cos(theta3).*sin(theta1).*sin(theta2).*1.0425e-2+sin(theta1).*sin(theta2).*sin(theta3).*2.67415e-8-cos(theta2).*cos(theta3).*sin(theta1).*2.67415e-8))))./2.0+(sin(theta1).*(-(cos(theta2).*sin(theta3)+cos(theta3).*sin(theta2)).*(sin(theta1).*(-2.74946e-3)+cos(theta1).*sin(theta2).*sin(theta3).*2.67415e-8-cos(theta1).*cos(theta2).*cos(theta3).*2.67415e-8+cos(theta1).*cos(theta2).*sin(theta3).*1.0425e-2+cos(theta1).*cos(theta3).*sin(theta2).*1.0425e-2)+(cos(theta2).*cos(theta3)-sin(theta2).*sin(theta3)).*(sin(theta1).*(-2.13561e-9)+cos(theta1).*sin(theta2).*sin(theta3).*7.5434e-2-cos(theta1).*cos(theta2).*cos(theta3).*7.5434e-2+cos(theta1).*cos(theta2).*sin(theta3).*2.67415e-8+cos(theta1).*cos(theta3).*sin(theta2).*2.67415e-8)+(cos(theta2).*cos(theta3)-sin(theta2).*sin(theta3)).*(cos(theta1).*sin(theta2).*sin(theta3).*(-1.0425e-2)+cos(theta1).*cos(theta2).*cos(theta3).*1.0425e-2+cos(theta1).*cos(theta2).*sin(theta3).*2.67415e-8+cos(theta1).*cos(theta3).*sin(theta2).*2.67415e-8)+(cos(theta2).*sin(theta3)+cos(theta3).*sin(theta2)).*(cos(theta1).*sin(theta2).*sin(theta3).*(-2.67415e-8)+cos(theta1).*cos(theta2).*cos(theta3).*2.67415e-8+cos(theta1).*cos(theta2).*sin(theta3).*7.5434e-2+cos(theta1).*cos(theta3).*sin(theta2).*7.5434e-2)))./2.0+(cos(theta1).*(cos(theta1).*(-sin(theta1).*(cos(theta1).*7.44749e-2+cos(theta2).*sin(theta1).*sin(theta3).*2.74946e-3+cos(theta3).*sin(theta1).*sin(theta2).*2.74946e-3+sin(theta1).*sin(theta2).*sin(theta3).*2.13561e-9-cos(theta2).*cos(theta3).*sin(theta1).*2.13561e-9)+(cos(theta1).*sin(theta2).*sin(theta3)-cos(theta1).*cos(theta2).*cos(theta3)).*(cos(theta1).*2.13561e-9+cos(theta2).*sin(theta1).*sin(theta3).*2.67415e-8+cos(theta3).*sin(theta1).*sin(theta2).*2.67415e-8+sin(theta1).*sin(theta2).*sin(theta3).*7.5434e-2-cos(theta2).*cos(theta3).*sin(theta1).*7.5434e-2)+(cos(theta1).*cos(theta2).*sin(theta3)+cos(theta1).*cos(theta3).*sin(theta2)).*(cos(theta1).*2.74946e-3+cos(theta2).*sin(theta1).*sin(theta3).*1.0425e-2+cos(theta3).*sin(theta1).*sin(theta2).*1.0425e-2+sin(theta1).*sin(theta2).*sin(theta3).*2.67415e-8-cos(theta2).*cos(theta3).*sin(theta1).*2.67415e-8))-sin(theta1).*(-sin(theta1).*(sin(theta1).*(-7.44749e-2)+cos(theta1).*sin(theta2).*sin(theta3).*2.13561e-9-cos(theta1).*cos(theta2).*cos(theta3).*2.13561e-9+cos(theta1).*cos(theta2).*sin(theta3).*2.74946e-3+cos(theta1).*cos(theta3).*sin(theta2).*2.74946e-3)+(cos(theta1).*sin(theta2).*sin(theta3)-cos(theta1).*cos(theta2).*cos(theta3)).*(sin(theta1).*(-2.13561e-9)+cos(theta1).*sin(theta2).*sin(theta3).*7.5434e-2-cos(theta1).*cos(theta2).*cos(theta3).*7.5434e-2+cos(theta1).*cos(theta2).*sin(theta3).*2.67415e-8+cos(theta1).*cos(theta3).*sin(theta2).*2.67415e-8)+(cos(theta1).*cos(theta2).*sin(theta3)+cos(theta1).*cos(theta3).*sin(theta2)).*(sin(theta1).*(-2.74946e-3)+cos(theta1).*sin(theta2).*sin(theta3).*2.67415e-8-cos(theta1).*cos(theta2).*cos(theta3).*2.67415e-8+cos(theta1).*cos(theta2).*sin(theta3).*1.0425e-2+cos(theta1).*cos(theta3).*sin(theta2).*1.0425e-2))))./2.0),theta3_dot.*(((cos(theta2).*sin(theta1).*sin(theta3).*1.20975e-1+cos(theta3).*sin(theta1).*sin(theta2).*1.20975e-1).*(sin(theta1).*sin(theta2).*sin(theta3).*6.228833385e-1-cos(theta2).*cos(theta3).*sin(theta1).*6.228833385e-1))./2.0+((sin(theta1).*sin(theta2).*sin(theta3).*1.20975e-1-cos(theta2).*cos(theta3).*sin(theta1).*1.20975e-1).*(cos(theta2).*sin(theta1).*sin(theta3).*6.228833385e-1+cos(theta3).*sin(theta1).*sin(theta2).*6.228833385e-1))./2.0+((cos(theta2).*cos(theta3).*1.20975e-1-sin(theta2).*sin(theta3).*1.20975e-1).*(cos(theta2).*sin(theta3).*6.228833385e-1+cos(theta3).*sin(theta2).*6.228833385e-1))./2.0+((cos(theta2).*sin(theta3).*1.20975e-1+cos(theta3).*sin(theta2).*1.20975e-1).*(cos(theta2).*cos(theta3).*6.228833385e-1-sin(theta2).*sin(theta3).*6.228833385e-1))./2.0-(cos(theta1).*(sin(theta1).*(cos(theta1).*(cos(theta1).*sin(theta2).*sin(theta3).*(-2.74946e-3)+cos(theta1).*cos(theta2).*cos(theta3).*2.74946e-3+cos(theta1).*cos(theta2).*sin(theta3).*2.13561e-9+cos(theta1).*cos(theta3).*sin(theta2).*2.13561e-9)+(cos(theta2).*sin(theta1).*sin(theta3)+cos(theta3).*sin(theta1).*sin(theta2)).*(sin(theta1).*(-2.13561e-9)+cos(theta1).*sin(theta2).*sin(theta3).*7.5434e-2-cos(theta1).*cos(theta2).*cos(theta3).*7.5434e-2+cos(theta1).*cos(theta2).*sin(theta3).*2.67415e-8+cos(theta1).*cos(theta3).*sin(theta2).*2.67415e-8)+(cos(theta2).*sin(theta1).*sin(theta3)+cos(theta3).*sin(theta1).*sin(theta2)).*(cos(theta1).*sin(theta2).*sin(theta3).*(-1.0425e-2)+cos(theta1).*cos(theta2).*cos(theta3).*1.0425e-2+cos(theta1).*cos(theta2).*sin(theta3).*2.67415e-8+cos(theta1).*cos(theta3).*sin(theta2).*2.67415e-8)+(sin(theta1).*sin(theta2).*sin(theta3)-cos(theta2).*cos(theta3).*sin(theta1)).*(cos(theta1).*sin(theta2).*sin(theta3).*(-2.67415e-8)+cos(theta1).*cos(theta2).*cos(theta3).*2.67415e-8+cos(theta1).*cos(theta2).*sin(theta3).*7.5434e-2+cos(theta1).*cos(theta3).*sin(theta2).*7.5434e-2)-(sin(theta1).*sin(theta2).*sin(theta3)-cos(theta2).*cos(theta3).*sin(theta1)).*(sin(theta1).*(-2.74946e-3)+cos(theta1).*sin(theta2).*sin(theta3).*2.67415e-8-cos(theta1).*cos(theta2).*cos(theta3).*2.67415e-8+cos(theta1).*cos(theta2).*sin(theta3).*1.0425e-2+cos(theta1).*cos(theta3).*sin(theta2).*1.0425e-2))-cos(theta1).*((sin(theta1).*sin(theta2).*sin(theta3)-cos(theta2).*cos(theta3).*sin(theta1)).*(cos(theta2).*sin(theta1).*sin(theta3).*7.5434e-2+cos(theta3).*sin(theta1).*sin(theta2).*7.5434e-2-sin(theta1).*sin(theta2).*sin(theta3).*2.67415e-8+cos(theta2).*cos(theta3).*sin(theta1).*2.67415e-8)-(sin(theta1).*sin(theta2).*sin(theta3)-cos(theta2).*cos(theta3).*sin(theta1)).*(cos(theta1).*2.74946e-3+cos(theta2).*sin(theta1).*sin(theta3).*1.0425e-2+cos(theta3).*sin(theta1).*sin(theta2).*1.0425e-2+sin(theta1).*sin(theta2).*sin(theta3).*2.67415e-8-cos(theta2).*cos(theta3).*sin(theta1).*2.67415e-8)+(cos(theta2).*sin(theta1).*sin(theta3)+cos(theta3).*sin(theta1).*sin(theta2)).*(cos(theta1).*2.13561e-9+cos(theta2).*sin(theta1).*sin(theta3).*2.67415e-8+cos(theta3).*sin(theta1).*sin(theta2).*2.67415e-8+sin(theta1).*sin(theta2).*sin(theta3).*7.5434e-2-cos(theta2).*cos(theta3).*sin(theta1).*7.5434e-2)+cos(theta1).*(cos(theta2).*sin(theta1).*sin(theta3).*2.13561e-9+cos(theta3).*sin(theta1).*sin(theta2).*2.13561e-9-sin(theta1).*sin(theta2).*sin(theta3).*2.74946e-3+cos(theta2).*cos(theta3).*sin(theta1).*2.74946e-3)+(cos(theta2).*sin(theta1).*sin(theta3)+cos(theta3).*sin(theta1).*sin(theta2)).*(cos(theta2).*sin(theta1).*sin(theta3).*2.67415e-8+cos(theta3).*sin(theta1).*sin(theta2).*2.67415e-8-sin(theta1).*sin(theta2).*sin(theta3).*1.0425e-2+cos(theta2).*cos(theta3).*sin(theta1).*1.0425e-2))))./2.0+(sin(theta1).*(sin(theta1).*((cos(theta1).*cos(theta2).*sin(theta3)+cos(theta1).*cos(theta3).*sin(theta2)).*(sin(theta1).*(-2.13561e-9)+cos(theta1).*sin(theta2).*sin(theta3).*7.5434e-2-cos(theta1).*cos(theta2).*cos(theta3).*7.5434e-2+cos(theta1).*cos(theta2).*sin(theta3).*2.67415e-8+cos(theta1).*cos(theta3).*sin(theta2).*2.67415e-8)+(cos(theta1).*cos(theta2).*sin(theta3)+cos(theta1).*cos(theta3).*sin(theta2)).*(cos(theta1).*sin(theta2).*sin(theta3).*(-1.0425e-2)+cos(theta1).*cos(theta2).*cos(theta3).*1.0425e-2+cos(theta1).*cos(theta2).*sin(theta3).*2.67415e-8+cos(theta1).*cos(theta3).*sin(theta2).*2.67415e-8)-sin(theta1).*(cos(theta1).*sin(theta2).*sin(theta3).*(-2.74946e-3)+cos(theta1).*cos(theta2).*cos(theta3).*2.74946e-3+cos(theta1).*cos(theta2).*sin(theta3).*2.13561e-9+cos(theta1).*cos(theta3).*sin(theta2).*2.13561e-9)+(cos(theta1).*sin(theta2).*sin(theta3)-cos(theta1).*cos(theta2).*cos(theta3)).*(cos(theta1).*sin(theta2).*sin(theta3).*(-2.67415e-8)+cos(theta1).*cos(theta2).*cos(theta3).*2.67415e-8+cos(theta1).*cos(theta2).*sin(theta3).*7.5434e-2+cos(theta1).*cos(theta3).*sin(theta2).*7.5434e-2)-(cos(theta1).*sin(theta2).*sin(theta3)-cos(theta1).*cos(theta2).*cos(theta3)).*(sin(theta1).*(-2.74946e-3)+cos(theta1).*sin(theta2).*sin(theta3).*2.67415e-8-cos(theta1).*cos(theta2).*cos(theta3).*2.67415e-8+cos(theta1).*cos(theta2).*sin(theta3).*1.0425e-2+cos(theta1).*cos(theta3).*sin(theta2).*1.0425e-2))-cos(theta1).*((cos(theta1).*cos(theta2).*sin(theta3)+cos(theta1).*cos(theta3).*sin(theta2)).*(cos(theta1).*2.13561e-9+cos(theta2).*sin(theta1).*sin(theta3).*2.67415e-8+cos(theta3).*sin(theta1).*sin(theta2).*2.67415e-8+sin(theta1).*sin(theta2).*sin(theta3).*7.5434e-2-cos(theta2).*cos(theta3).*sin(theta1).*7.5434e-2)+(cos(theta1).*cos(theta2).*sin(theta3)+cos(theta1).*cos(theta3).*sin(theta2)).*(cos(theta2).*sin(theta1).*sin(theta3).*2.67415e-8+cos(theta3).*sin(theta1).*sin(theta2).*2.67415e-8-sin(theta1).*sin(theta2).*sin(theta3).*1.0425e-2+cos(theta2).*cos(theta3).*sin(theta1).*1.0425e-2)-sin(theta1).*(cos(theta2).*sin(theta1).*sin(theta3).*2.13561e-9+cos(theta3).*sin(theta1).*sin(theta2).*2.13561e-9-sin(theta1).*sin(theta2).*sin(theta3).*2.74946e-3+cos(theta2).*cos(theta3).*sin(theta1).*2.74946e-3)+(cos(theta1).*sin(theta2).*sin(theta3)-cos(theta1).*cos(theta2).*cos(theta3)).*(cos(theta2).*sin(theta1).*sin(theta3).*7.5434e-2+cos(theta3).*sin(theta1).*sin(theta2).*7.5434e-2-sin(theta1).*sin(theta2).*sin(theta3).*2.67415e-8+cos(theta2).*cos(theta3).*sin(theta1).*2.67415e-8)-(cos(theta1).*sin(theta2).*sin(theta3)-cos(theta1).*cos(theta2).*cos(theta3)).*(cos(theta1).*2.74946e-3+cos(theta2).*sin(theta1).*sin(theta3).*1.0425e-2+cos(theta3).*sin(theta1).*sin(theta2).*1.0425e-2+sin(theta1).*sin(theta2).*sin(theta3).*2.67415e-8-cos(theta2).*cos(theta3).*sin(theta1).*2.67415e-8))))./2.0+((cos(theta1).*sin(theta2).*sin(theta3).*1.20975e-1-cos(theta1).*cos(theta2).*cos(theta3).*1.20975e-1).*(cos(theta1).*cos(theta2).*sin(theta3).*6.228833385e-1+cos(theta1).*cos(theta3).*sin(theta2).*6.228833385e-1))./2.0+((cos(theta1).*cos(theta2).*sin(theta3).*1.20975e-1+cos(theta1).*cos(theta3).*sin(theta2).*1.20975e-1).*(cos(theta1).*sin(theta2).*sin(theta3).*6.228833385e-1-cos(theta1).*cos(theta2).*cos(theta3).*6.228833385e-1))./2.0)-theta1_dot.*((cos(theta1).*(cos(theta1).*(cos(theta1).*(sin(theta1).*(-7.44749e-2)+cos(theta1).*sin(theta2).*sin(theta3).*2.13561e-9-cos(theta1).*cos(theta2).*cos(theta3).*2.13561e-9+cos(theta1).*cos(theta2).*sin(theta3).*2.74946e-3+cos(theta1).*cos(theta3).*sin(theta2).*2.74946e-3)+(sin(theta1).*sin(theta2).*sin(theta3)-cos(theta2).*cos(theta3).*sin(theta1)).*(sin(theta1).*(-2.13561e-9)+cos(theta1).*sin(theta2).*sin(theta3).*7.5434e-2-cos(theta1).*cos(theta2).*cos(theta3).*7.5434e-2+cos(theta1).*cos(theta2).*sin(theta3).*2.67415e-8+cos(theta1).*cos(theta3).*sin(theta2).*2.67415e-8)+(cos(theta2).*sin(theta1).*sin(theta3)+cos(theta3).*sin(theta1).*sin(theta2)).*(sin(theta1).*(-2.74946e-3)+cos(theta1).*sin(theta2).*sin(theta3).*2.67415e-8-cos(theta1).*cos(theta2).*cos(theta3).*2.67415e-8+cos(theta1).*cos(theta2).*sin(theta3).*1.0425e-2+cos(theta1).*cos(theta3).*sin(theta2).*1.0425e-2))+sin(theta1).*((cos(theta2).*sin(theta1).*sin(theta3)+cos(theta3).*sin(theta1).*sin(theta2)).*(cos(theta1).*2.74946e-3+cos(theta2).*sin(theta1).*sin(theta3).*1.0425e-2+cos(theta3).*sin(theta1).*sin(theta2).*1.0425e-2+sin(theta1).*sin(theta2).*sin(theta3).*2.67415e-8-cos(theta2).*cos(theta3).*sin(theta1).*2.67415e-8)+cos(theta1).*(cos(theta1).*7.44749e-2+cos(theta2).*sin(theta1).*sin(theta3).*2.74946e-3+cos(theta3).*sin(theta1).*sin(theta2).*2.74946e-3+sin(theta1).*sin(theta2).*sin(theta3).*2.13561e-9-cos(theta2).*cos(theta3).*sin(theta1).*2.13561e-9)+(sin(theta1).*sin(theta2).*sin(theta3)-cos(theta2).*cos(theta3).*sin(theta1)).*(cos(theta1).*2.13561e-9+cos(theta2).*sin(theta1).*sin(theta3).*2.67415e-8+cos(theta3).*sin(theta1).*sin(theta2).*2.67415e-8+sin(theta1).*sin(theta2).*sin(theta3).*7.5434e-2-cos(theta2).*cos(theta3).*sin(theta1).*7.5434e-2))-cos(theta1).*(cos(theta1).*(sin(theta1).*(-7.44749e-2)+cos(theta1).*sin(theta2).*sin(theta3).*2.13561e-9-cos(theta1).*cos(theta2).*cos(theta3).*2.13561e-9+cos(theta1).*cos(theta2).*sin(theta3).*2.74946e-3+cos(theta1).*cos(theta3).*sin(theta2).*2.74946e-3)+(sin(theta1).*sin(theta2).*sin(theta3)-cos(theta2).*cos(theta3).*sin(theta1)).*(sin(theta1).*(-2.13561e-9)+cos(theta1).*sin(theta2).*sin(theta3).*7.5434e-2-cos(theta1).*cos(theta2).*cos(theta3).*7.5434e-2+cos(theta1).*cos(theta2).*sin(theta3).*2.67415e-8+cos(theta1).*cos(theta3).*sin(theta2).*2.67415e-8)-sin(theta1).*(cos(theta1).*7.44749e-2+cos(theta2).*sin(theta1).*sin(theta3).*2.74946e-3+cos(theta3).*sin(theta1).*sin(theta2).*2.74946e-3+sin(theta1).*sin(theta2).*sin(theta3).*2.13561e-9-cos(theta2).*cos(theta3).*sin(theta1).*2.13561e-9)+(cos(theta1).*sin(theta2).*sin(theta3)-cos(theta1).*cos(theta2).*cos(theta3)).*(cos(theta1).*2.13561e-9+cos(theta2).*sin(theta1).*sin(theta3).*2.67415e-8+cos(theta3).*sin(theta1).*sin(theta2).*2.67415e-8+sin(theta1).*sin(theta2).*sin(theta3).*7.5434e-2-cos(theta2).*cos(theta3).*sin(theta1).*7.5434e-2)+(cos(theta2).*sin(theta1).*sin(theta3)+cos(theta3).*sin(theta1).*sin(theta2)).*(sin(theta1).*(-2.74946e-3)+cos(theta1).*sin(theta2).*sin(theta3).*2.67415e-8-cos(theta1).*cos(theta2).*cos(theta3).*2.67415e-8+cos(theta1).*cos(theta2).*sin(theta3).*1.0425e-2+cos(theta1).*cos(theta3).*sin(theta2).*1.0425e-2)+(cos(theta1).*cos(theta2).*sin(theta3)+cos(theta1).*cos(theta3).*sin(theta2)).*(cos(theta1).*2.74946e-3+cos(theta2).*sin(theta1).*sin(theta3).*1.0425e-2+cos(theta3).*sin(theta1).*sin(theta2).*1.0425e-2+sin(theta1).*sin(theta2).*sin(theta3).*2.67415e-8-cos(theta2).*cos(theta3).*sin(theta1).*2.67415e-8))-sin(theta1).*((cos(theta2).*sin(theta1).*sin(theta3)+cos(theta3).*sin(theta1).*sin(theta2)).*(cos(theta1).*2.74946e-3+cos(theta2).*sin(theta1).*sin(theta3).*1.0425e-2+cos(theta3).*sin(theta1).*sin(theta2).*1.0425e-2+sin(theta1).*sin(theta2).*sin(theta3).*2.67415e-8-cos(theta2).*cos(theta3).*sin(theta1).*2.67415e-8)+sin(theta1).*(sin(theta1).*(-7.44749e-2)+cos(theta1).*sin(theta2).*sin(theta3).*2.13561e-9-cos(theta1).*cos(theta2).*cos(theta3).*2.13561e-9+cos(theta1).*cos(theta2).*sin(theta3).*2.74946e-3+cos(theta1).*cos(theta3).*sin(theta2).*2.74946e-3)-(cos(theta1).*sin(theta2).*sin(theta3)-cos(theta1).*cos(theta2).*cos(theta3)).*(sin(theta1).*(-2.13561e-9)+cos(theta1).*sin(theta2).*sin(theta3).*7.5434e-2-cos(theta1).*cos(theta2).*cos(theta3).*7.5434e-2+cos(theta1).*cos(theta2).*sin(theta3).*2.67415e-8+cos(theta1).*cos(theta3).*sin(theta2).*2.67415e-8)+cos(theta1).*(cos(theta1).*7.44749e-2+cos(theta2).*sin(theta1).*sin(theta3).*2.74946e-3+cos(theta3).*sin(theta1).*sin(theta2).*2.74946e-3+sin(theta1).*sin(theta2).*sin(theta3).*2.13561e-9-cos(theta2).*cos(theta3).*sin(theta1).*2.13561e-9)+(sin(theta1).*sin(theta2).*sin(theta3)-cos(theta2).*cos(theta3).*sin(theta1)).*(cos(theta1).*2.13561e-9+cos(theta2).*sin(theta1).*sin(theta3).*2.67415e-8+cos(theta3).*sin(theta1).*sin(theta2).*2.67415e-8+sin(theta1).*sin(theta2).*sin(theta3).*7.5434e-2-cos(theta2).*cos(theta3).*sin(theta1).*7.5434e-2)-(cos(theta1).*cos(theta2).*sin(theta3)+cos(theta1).*cos(theta3).*sin(theta2)).*(sin(theta1).*(-2.74946e-3)+cos(theta1).*sin(theta2).*sin(theta3).*2.67415e-8-cos(theta1).*cos(theta2).*cos(theta3).*2.67415e-8+cos(theta1).*cos(theta2).*sin(theta3).*1.0425e-2+cos(theta1).*cos(theta3).*sin(theta2).*1.0425e-2))))./2.0-(cos(theta1).*sin(theta2).*sin(theta3).*1.20975e-1-cos(theta1).*cos(theta2).*cos(theta3).*1.20975e-1).*(sin(theta1).*sin(theta2).*sin(theta3).*6.228833385e-1-cos(theta2).*cos(theta3).*sin(theta1).*6.228833385e-1)+(cos(theta1).*sin(theta2).*sin(theta3).*6.228833385e-1-cos(theta1).*cos(theta2).*cos(theta3).*6.228833385e-1).*(sin(theta1).*sin(theta2).*sin(theta3).*1.20975e-1-cos(theta2).*cos(theta3).*sin(theta1).*1.20975e-1)+((cos(theta1).*cos(theta2).*sin(theta3).*1.20975e-1+cos(theta1).*cos(theta3).*sin(theta2).*1.20975e-1).*(cos(theta1).*2.272809781200003e-2+sin(theta1).*sin(theta2).*2.2140098+cos(theta2).*sin(theta1).*sin(theta3).*6.228833385e-1+cos(theta3).*sin(theta1).*sin(theta2).*6.228833385e-1))./2.0-((cos(theta2).*sin(theta1).*sin(theta3).*1.20975e-1+cos(theta3).*sin(theta1).*sin(theta2).*1.20975e-1).*(sin(theta1).*(-2.272809781200003e-2)+cos(theta1).*sin(theta2).*2.2140098+cos(theta1).*cos(theta2).*sin(theta3).*6.228833385e-1+cos(theta1).*cos(theta3).*sin(theta2).*6.228833385e-1))./2.0-((cos(theta1).*cos(theta2).*sin(theta3).*6.228833385e-1+cos(theta1).*cos(theta3).*sin(theta2).*6.228833385e-1).*(cos(theta1).*4.414200000000005e-3+sin(theta1).*sin(theta2).*(4.3e+1./1.0e+2)+cos(theta2).*sin(theta1).*sin(theta3).*1.20975e-1+cos(theta3).*sin(theta1).*sin(theta2).*1.20975e-1))./2.0+((cos(theta2).*sin(theta1).*sin(theta3).*6.228833385e-1+cos(theta3).*sin(theta1).*sin(theta2).*6.228833385e-1).*(sin(theta1).*(-4.414200000000005e-3)+cos(theta1).*sin(theta2).*(4.3e+1./1.0e+2)+cos(theta1).*cos(theta2).*sin(theta3).*1.20975e-1+cos(theta1).*cos(theta3).*sin(theta2).*1.20975e-1))./2.0+(sin(theta1).*(-sin(theta1).*(cos(theta2).*cos(theta3).*(-2.13561e-9)+cos(theta2).*sin(theta3).*2.74946e-3+cos(theta3).*sin(theta2).*2.74946e-3+sin(theta2).*sin(theta3).*2.13561e-9)-(cos(theta1).*cos(theta2).*sin(theta3)+cos(theta1).*cos(theta3).*sin(theta2)).*(cos(theta2).*cos(theta3).*2.67415e-8+cos(theta2).*sin(theta3).*7.5434e-2+cos(theta3).*sin(theta2).*7.5434e-2-sin(theta2).*sin(theta3).*2.67415e-8)+(cos(theta1).*sin(theta2).*sin(theta3)-cos(theta1).*cos(theta2).*cos(theta3)).*(cos(theta2).*cos(theta3).*(-7.5434e-2)+cos(theta2).*sin(theta3).*2.67415e-8+cos(theta3).*sin(theta2).*2.67415e-8+sin(theta2).*sin(theta3).*7.5434e-2)+(cos(theta1).*cos(theta2).*sin(theta3)+cos(theta1).*cos(theta3).*sin(theta2)).*(cos(theta2).*cos(theta3).*(-2.67415e-8)+cos(theta2).*sin(theta3).*1.0425e-2+cos(theta3).*sin(theta2).*1.0425e-2+sin(theta2).*sin(theta3).*2.67415e-8)+(cos(theta1).*sin(theta2).*sin(theta3)-cos(theta1).*cos(theta2).*cos(theta3)).*(cos(theta2).*cos(theta3).*1.0425e-2+cos(theta2).*sin(theta3).*2.67415e-8+cos(theta3).*sin(theta2).*2.67415e-8-sin(theta2).*sin(theta3).*1.0425e-2)))./2.0-(sin(theta1).*(sin(theta1).*(cos(theta1).*(sin(theta1).*(-7.44749e-2)+cos(theta1).*sin(theta2).*sin(theta3).*2.13561e-9-cos(theta1).*cos(theta2).*cos(theta3).*2.13561e-9+cos(theta1).*cos(theta2).*sin(theta3).*2.74946e-3+cos(theta1).*cos(theta3).*sin(theta2).*2.74946e-3)+(sin(theta1).*sin(theta2).*sin(theta3)-cos(theta2).*cos(theta3).*sin(theta1)).*(sin(theta1).*(-2.13561e-9)+cos(theta1).*sin(theta2).*sin(theta3).*7.5434e-2-cos(theta1).*cos(theta2).*cos(theta3).*7.5434e-2+cos(theta1).*cos(theta2).*sin(theta3).*2.67415e-8+cos(theta1).*cos(theta3).*sin(theta2).*2.67415e-8)+(cos(theta2).*sin(theta1).*sin(theta3)+cos(theta3).*sin(theta1).*sin(theta2)).*(sin(theta1).*(-2.74946e-3)+cos(theta1).*sin(theta2).*sin(theta3).*2.67415e-8-cos(theta1).*cos(theta2).*cos(theta3).*2.67415e-8+cos(theta1).*cos(theta2).*sin(theta3).*1.0425e-2+cos(theta1).*cos(theta3).*sin(theta2).*1.0425e-2))-cos(theta1).*((cos(theta2).*sin(theta1).*sin(theta3)+cos(theta3).*sin(theta1).*sin(theta2)).*(cos(theta1).*2.74946e-3+cos(theta2).*sin(theta1).*sin(theta3).*1.0425e-2+cos(theta3).*sin(theta1).*sin(theta2).*1.0425e-2+sin(theta1).*sin(theta2).*sin(theta3).*2.67415e-8-cos(theta2).*cos(theta3).*sin(theta1).*2.67415e-8)+cos(theta1).*(cos(theta1).*7.44749e-2+cos(theta2).*sin(theta1).*sin(theta3).*2.74946e-3+cos(theta3).*sin(theta1).*sin(theta2).*2.74946e-3+sin(theta1).*sin(theta2).*sin(theta3).*2.13561e-9-cos(theta2).*cos(theta3).*sin(theta1).*2.13561e-9)+(sin(theta1).*sin(theta2).*sin(theta3)-cos(theta2).*cos(theta3).*sin(theta1)).*(cos(theta1).*2.13561e-9+cos(theta2).*sin(theta1).*sin(theta3).*2.67415e-8+cos(theta3).*sin(theta1).*sin(theta2).*2.67415e-8+sin(theta1).*sin(theta2).*sin(theta3).*7.5434e-2-cos(theta2).*cos(theta3).*sin(theta1).*7.5434e-2))))./2.0-(cos(theta1).*(cos(theta1).*(cos(theta2).*cos(theta3).*(-2.13561e-9)+cos(theta2).*sin(theta3).*2.74946e-3+cos(theta3).*sin(theta2).*2.74946e-3+sin(theta2).*sin(theta3).*2.13561e-9)+(cos(theta2).*sin(theta1).*sin(theta3)+cos(theta3).*sin(theta1).*sin(theta2)).*(cos(theta2).*cos(theta3).*(-2.67415e-8)+cos(theta2).*sin(theta3).*1.0425e-2+cos(theta3).*sin(theta2).*1.0425e-2+sin(theta2).*sin(theta3).*2.67415e-8)+(sin(theta1).*sin(theta2).*sin(theta3)-cos(theta2).*cos(theta3).*sin(theta1)).*(cos(theta2).*cos(theta3).*1.0425e-2+cos(theta2).*sin(theta3).*2.67415e-8+cos(theta3).*sin(theta2).*2.67415e-8-sin(theta2).*sin(theta3).*1.0425e-2)-(cos(theta2).*sin(theta1).*sin(theta3)+cos(theta3).*sin(theta1).*sin(theta2)).*(cos(theta2).*cos(theta3).*2.67415e-8+cos(theta2).*sin(theta3).*7.5434e-2+cos(theta3).*sin(theta2).*7.5434e-2-sin(theta2).*sin(theta3).*2.67415e-8)+(sin(theta1).*sin(theta2).*sin(theta3)-cos(theta2).*cos(theta3).*sin(theta1)).*(cos(theta2).*cos(theta3).*(-7.5434e-2)+cos(theta2).*sin(theta3).*2.67415e-8+cos(theta3).*sin(theta2).*2.67415e-8+sin(theta2).*sin(theta3).*7.5434e-2)))./2.0-(cos(theta1).*((cos(theta2).*sin(theta3)+cos(theta3).*sin(theta2)).*(cos(theta2).*sin(theta1).*sin(theta3).*7.5434e-2+cos(theta3).*sin(theta1).*sin(theta2).*7.5434e-2-sin(theta1).*sin(theta2).*sin(theta3).*2.67415e-8+cos(theta2).*cos(theta3).*sin(theta1).*2.67415e-8)-(cos(theta2).*sin(theta3)+cos(theta3).*sin(theta2)).*(cos(theta1).*2.74946e-3+cos(theta2).*sin(theta1).*sin(theta3).*1.0425e-2+cos(theta3).*sin(theta1).*sin(theta2).*1.0425e-2+sin(theta1).*sin(theta2).*sin(theta3).*2.67415e-8-cos(theta2).*cos(theta3).*sin(theta1).*2.67415e-8)+(cos(theta2).*cos(theta3)-sin(theta2).*sin(theta3)).*(cos(theta1).*2.13561e-9+cos(theta2).*sin(theta1).*sin(theta3).*2.67415e-8+cos(theta3).*sin(theta1).*sin(theta2).*2.67415e-8+sin(theta1).*sin(theta2).*sin(theta3).*7.5434e-2-cos(theta2).*cos(theta3).*sin(theta1).*7.5434e-2)+(cos(theta2).*cos(theta3)-sin(theta2).*sin(theta3)).*(cos(theta2).*sin(theta1).*sin(theta3).*2.67415e-8+cos(theta3).*sin(theta1).*sin(theta2).*2.67415e-8-sin(theta1).*sin(theta2).*sin(theta3).*1.0425e-2+cos(theta2).*cos(theta3).*sin(theta1).*1.0425e-2)))./2.0-(sin(theta1).*(sin(theta1).*(-sin(theta1).*(cos(theta1).*7.44749e-2+cos(theta2).*sin(theta1).*sin(theta3).*2.74946e-3+cos(theta3).*sin(theta1).*sin(theta2).*2.74946e-3+sin(theta1).*sin(theta2).*sin(theta3).*2.13561e-9-cos(theta2).*cos(theta3).*sin(theta1).*2.13561e-9)+(cos(theta1).*sin(theta2).*sin(theta3)-cos(theta1).*cos(theta2).*cos(theta3)).*(cos(theta1).*2.13561e-9+cos(theta2).*sin(theta1).*sin(theta3).*2.67415e-8+cos(theta3).*sin(theta1).*sin(theta2).*2.67415e-8+sin(theta1).*sin(theta2).*sin(theta3).*7.5434e-2-cos(theta2).*cos(theta3).*sin(theta1).*7.5434e-2)+(cos(theta1).*cos(theta2).*sin(theta3)+cos(theta1).*cos(theta3).*sin(theta2)).*(cos(theta1).*2.74946e-3+cos(theta2).*sin(theta1).*sin(theta3).*1.0425e-2+cos(theta3).*sin(theta1).*sin(theta2).*1.0425e-2+sin(theta1).*sin(theta2).*sin(theta3).*2.67415e-8-cos(theta2).*cos(theta3).*sin(theta1).*2.67415e-8))+cos(theta1).*(-sin(theta1).*(sin(theta1).*(-7.44749e-2)+cos(theta1).*sin(theta2).*sin(theta3).*2.13561e-9-cos(theta1).*cos(theta2).*cos(theta3).*2.13561e-9+cos(theta1).*cos(theta2).*sin(theta3).*2.74946e-3+cos(theta1).*cos(theta3).*sin(theta2).*2.74946e-3)+(cos(theta1).*sin(theta2).*sin(theta3)-cos(theta1).*cos(theta2).*cos(theta3)).*(sin(theta1).*(-2.13561e-9)+cos(theta1).*sin(theta2).*sin(theta3).*7.5434e-2-cos(theta1).*cos(theta2).*cos(theta3).*7.5434e-2+cos(theta1).*cos(theta2).*sin(theta3).*2.67415e-8+cos(theta1).*cos(theta3).*sin(theta2).*2.67415e-8)+(cos(theta1).*cos(theta2).*sin(theta3)+cos(theta1).*cos(theta3).*sin(theta2)).*(sin(theta1).*(-2.74946e-3)+cos(theta1).*sin(theta2).*sin(theta3).*2.67415e-8-cos(theta1).*cos(theta2).*cos(theta3).*2.67415e-8+cos(theta1).*cos(theta2).*sin(theta3).*1.0425e-2+cos(theta1).*cos(theta3).*sin(theta2).*1.0425e-2))+cos(theta1).*((cos(theta2).*sin(theta1).*sin(theta3)+cos(theta3).*sin(theta1).*sin(theta2)).*(cos(theta1).*2.74946e-3+cos(theta2).*sin(theta1).*sin(theta3).*1.0425e-2+cos(theta3).*sin(theta1).*sin(theta2).*1.0425e-2+sin(theta1).*sin(theta2).*sin(theta3).*2.67415e-8-cos(theta2).*cos(theta3).*sin(theta1).*2.67415e-8)+sin(theta1).*(sin(theta1).*(-7.44749e-2)+cos(theta1).*sin(theta2).*sin(theta3).*2.13561e-9-cos(theta1).*cos(theta2).*cos(theta3).*2.13561e-9+cos(theta1).*cos(theta2).*sin(theta3).*2.74946e-3+cos(theta1).*cos(theta3).*sin(theta2).*2.74946e-3)-(cos(theta1).*sin(theta2).*sin(theta3)-cos(theta1).*cos(theta2).*cos(theta3)).*(sin(theta1).*(-2.13561e-9)+cos(theta1).*sin(theta2).*sin(theta3).*7.5434e-2-cos(theta1).*cos(theta2).*cos(theta3).*7.5434e-2+cos(theta1).*cos(theta2).*sin(theta3).*2.67415e-8+cos(theta1).*cos(theta3).*sin(theta2).*2.67415e-8)+cos(theta1).*(cos(theta1).*7.44749e-2+cos(theta2).*sin(theta1).*sin(theta3).*2.74946e-3+cos(theta3).*sin(theta1).*sin(theta2).*2.74946e-3+sin(theta1).*sin(theta2).*sin(theta3).*2.13561e-9-cos(theta2).*cos(theta3).*sin(theta1).*2.13561e-9)+(sin(theta1).*sin(theta2).*sin(theta3)-cos(theta2).*cos(theta3).*sin(theta1)).*(cos(theta1).*2.13561e-9+cos(theta2).*sin(theta1).*sin(theta3).*2.67415e-8+cos(theta3).*sin(theta1).*sin(theta2).*2.67415e-8+sin(theta1).*sin(theta2).*sin(theta3).*7.5434e-2-cos(theta2).*cos(theta3).*sin(theta1).*7.5434e-2)-(cos(theta1).*cos(theta2).*sin(theta3)+cos(theta1).*cos(theta3).*sin(theta2)).*(sin(theta1).*(-2.74946e-3)+cos(theta1).*sin(theta2).*sin(theta3).*2.67415e-8-cos(theta1).*cos(theta2).*cos(theta3).*2.67415e-8+cos(theta1).*cos(theta2).*sin(theta3).*1.0425e-2+cos(theta1).*cos(theta3).*sin(theta2).*1.0425e-2))-sin(theta1).*(cos(theta1).*(sin(theta1).*(-7.44749e-2)+cos(theta1).*sin(theta2).*sin(theta3).*2.13561e-9-cos(theta1).*cos(theta2).*cos(theta3).*2.13561e-9+cos(theta1).*cos(theta2).*sin(theta3).*2.74946e-3+cos(theta1).*cos(theta3).*sin(theta2).*2.74946e-3)+(sin(theta1).*sin(theta2).*sin(theta3)-cos(theta2).*cos(theta3).*sin(theta1)).*(sin(theta1).*(-2.13561e-9)+cos(theta1).*sin(theta2).*sin(theta3).*7.5434e-2-cos(theta1).*cos(theta2).*cos(theta3).*7.5434e-2+cos(theta1).*cos(theta2).*sin(theta3).*2.67415e-8+cos(theta1).*cos(theta3).*sin(theta2).*2.67415e-8)-sin(theta1).*(cos(theta1).*7.44749e-2+cos(theta2).*sin(theta1).*sin(theta3).*2.74946e-3+cos(theta3).*sin(theta1).*sin(theta2).*2.74946e-3+sin(theta1).*sin(theta2).*sin(theta3).*2.13561e-9-cos(theta2).*cos(theta3).*sin(theta1).*2.13561e-9)+(cos(theta1).*sin(theta2).*sin(theta3)-cos(theta1).*cos(theta2).*cos(theta3)).*(cos(theta1).*2.13561e-9+cos(theta2).*sin(theta1).*sin(theta3).*2.67415e-8+cos(theta3).*sin(theta1).*sin(theta2).*2.67415e-8+sin(theta1).*sin(theta2).*sin(theta3).*7.5434e-2-cos(theta2).*cos(theta3).*sin(theta1).*7.5434e-2)+(cos(theta2).*sin(theta1).*sin(theta3)+cos(theta3).*sin(theta1).*sin(theta2)).*(sin(theta1).*(-2.74946e-3)+cos(theta1).*sin(theta2).*sin(theta3).*2.67415e-8-cos(theta1).*cos(theta2).*cos(theta3).*2.67415e-8+cos(theta1).*cos(theta2).*sin(theta3).*1.0425e-2+cos(theta1).*cos(theta3).*sin(theta2).*1.0425e-2)+(cos(theta1).*cos(theta2).*sin(theta3)+cos(theta1).*cos(theta3).*sin(theta2)).*(cos(theta1).*2.74946e-3+cos(theta2).*sin(theta1).*sin(theta3).*1.0425e-2+cos(theta3).*sin(theta1).*sin(theta2).*1.0425e-2+sin(theta1).*sin(theta2).*sin(theta3).*2.67415e-8-cos(theta2).*cos(theta3).*sin(theta1).*2.67415e-8))))./2.0+(sin(theta1).*(-(cos(theta2).*sin(theta3)+cos(theta3).*sin(theta2)).*(sin(theta1).*(-2.74946e-3)+cos(theta1).*sin(theta2).*sin(theta3).*2.67415e-8-cos(theta1).*cos(theta2).*cos(theta3).*2.67415e-8+cos(theta1).*cos(theta2).*sin(theta3).*1.0425e-2+cos(theta1).*cos(theta3).*sin(theta2).*1.0425e-2)+(cos(theta2).*cos(theta3)-sin(theta2).*sin(theta3)).*(sin(theta1).*(-2.13561e-9)+cos(theta1).*sin(theta2).*sin(theta3).*7.5434e-2-cos(theta1).*cos(theta2).*cos(theta3).*7.5434e-2+cos(theta1).*cos(theta2).*sin(theta3).*2.67415e-8+cos(theta1).*cos(theta3).*sin(theta2).*2.67415e-8)+(cos(theta2).*cos(theta3)-sin(theta2).*sin(theta3)).*(cos(theta1).*sin(theta2).*sin(theta3).*(-1.0425e-2)+cos(theta1).*cos(theta2).*cos(theta3).*1.0425e-2+cos(theta1).*cos(theta2).*sin(theta3).*2.67415e-8+cos(theta1).*cos(theta3).*sin(theta2).*2.67415e-8)+(cos(theta2).*sin(theta3)+cos(theta3).*sin(theta2)).*(cos(theta1).*sin(theta2).*sin(theta3).*(-2.67415e-8)+cos(theta1).*cos(theta2).*cos(theta3).*2.67415e-8+cos(theta1).*cos(theta2).*sin(theta3).*7.5434e-2+cos(theta1).*cos(theta3).*sin(theta2).*7.5434e-2)))./2.0+(cos(theta1).*(cos(theta1).*(-sin(theta1).*(cos(theta1).*7.44749e-2+cos(theta2).*sin(theta1).*sin(theta3).*2.74946e-3+cos(theta3).*sin(theta1).*sin(theta2).*2.74946e-3+sin(theta1).*sin(theta2).*sin(theta3).*2.13561e-9-cos(theta2).*cos(theta3).*sin(theta1).*2.13561e-9)+(cos(theta1).*sin(theta2).*sin(theta3)-cos(theta1).*cos(theta2).*cos(theta3)).*(cos(theta1).*2.13561e-9+cos(theta2).*sin(theta1).*sin(theta3).*2.67415e-8+cos(theta3).*sin(theta1).*sin(theta2).*2.67415e-8+sin(theta1).*sin(theta2).*sin(theta3).*7.5434e-2-cos(theta2).*cos(theta3).*sin(theta1).*7.5434e-2)+(cos(theta1).*cos(theta2).*sin(theta3)+cos(theta1).*cos(theta3).*sin(theta2)).*(cos(theta1).*2.74946e-3+cos(theta2).*sin(theta1).*sin(theta3).*1.0425e-2+cos(theta3).*sin(theta1).*sin(theta2).*1.0425e-2+sin(theta1).*sin(theta2).*sin(theta3).*2.67415e-8-cos(theta2).*cos(theta3).*sin(theta1).*2.67415e-8))-sin(theta1).*(-sin(theta1).*(sin(theta1).*(-7.44749e-2)+cos(theta1).*sin(theta2).*sin(theta3).*2.13561e-9-cos(theta1).*cos(theta2).*cos(theta3).*2.13561e-9+cos(theta1).*cos(theta2).*sin(theta3).*2.74946e-3+cos(theta1).*cos(theta3).*sin(theta2).*2.74946e-3)+(cos(theta1).*sin(theta2).*sin(theta3)-cos(theta1).*cos(theta2).*cos(theta3)).*(sin(theta1).*(-2.13561e-9)+cos(theta1).*sin(theta2).*sin(theta3).*7.5434e-2-cos(theta1).*cos(theta2).*cos(theta3).*7.5434e-2+cos(theta1).*cos(theta2).*sin(theta3).*2.67415e-8+cos(theta1).*cos(theta3).*sin(theta2).*2.67415e-8)+(cos(theta1).*cos(theta2).*sin(theta3)+cos(theta1).*cos(theta3).*sin(theta2)).*(sin(theta1).*(-2.74946e-3)+cos(theta1).*sin(theta2).*sin(theta3).*2.67415e-8-cos(theta1).*cos(theta2).*cos(theta3).*2.67415e-8+cos(theta1).*cos(theta2).*sin(theta3).*1.0425e-2+cos(theta1).*cos(theta3).*sin(theta2).*1.0425e-2))))./2.0)+theta2_dot.*((cos(theta1).*cos(theta2).*sin(theta3).*6.228833385e-1+cos(theta1).*cos(theta3).*sin(theta2).*6.228833385e-1).*(cos(theta1).*cos(theta2).*(4.3e+1./1.0e+2)-cos(theta1).*sin(theta2).*sin(theta3).*1.20975e-1+cos(theta1).*cos(theta2).*cos(theta3).*1.20975e-1).*(-1.0./2.0)+(cos(theta2).*sin(theta1).*sin(theta3).*1.20975e-1+cos(theta3).*sin(theta1).*sin(theta2).*1.20975e-1).*(sin(theta1).*sin(theta2).*sin(theta3).*6.228833385e-1-cos(theta2).*cos(theta3).*sin(theta1).*6.228833385e-1)-((cos(theta2).*sin(theta1).*sin(theta3).*6.228833385e-1+cos(theta3).*sin(theta1).*sin(theta2).*6.228833385e-1).*(cos(theta2).*sin(theta1).*(4.3e+1./1.0e+2)-sin(theta1).*sin(theta2).*sin(theta3).*1.20975e-1+cos(theta2).*cos(theta3).*sin(theta1).*1.20975e-1))./2.0-((cos(theta2).*cos(theta3).*1.20975e-1-sin(theta2).*sin(theta3).*1.20975e-1).*(sin(theta2).*2.2140098+cos(theta2).*sin(theta3).*6.228833385e-1+cos(theta3).*sin(theta2).*6.228833385e-1))./2.0+((cos(theta1).*cos(theta2).*sin(theta3).*1.20975e-1+cos(theta1).*cos(theta3).*sin(theta2).*1.20975e-1).*(cos(theta1).*cos(theta2).*2.2140098-cos(theta1).*sin(theta2).*sin(theta3).*6.228833385e-1+cos(theta1).*cos(theta2).*cos(theta3).*6.228833385e-1))./2.0+(cos(theta2).*cos(theta3).*1.20975e-1-sin(theta2).*sin(theta3).*1.20975e-1).*(cos(theta2).*sin(theta3).*6.228833385e-1+cos(theta3).*sin(theta2).*6.228833385e-1)-(cos(theta1).*(sin(theta1).*(cos(theta1).*(cos(theta1).*sin(theta2).*sin(theta3).*(-2.74946e-3)+cos(theta1).*cos(theta2).*cos(theta3).*2.74946e-3+cos(theta1).*cos(theta2).*sin(theta3).*2.13561e-9+cos(theta1).*cos(theta3).*sin(theta2).*2.13561e-9)+(cos(theta2).*sin(theta1).*sin(theta3)+cos(theta3).*sin(theta1).*sin(theta2)).*(sin(theta1).*(-2.13561e-9)+cos(theta1).*sin(theta2).*sin(theta3).*7.5434e-2-cos(theta1).*cos(theta2).*cos(theta3).*7.5434e-2+cos(theta1).*cos(theta2).*sin(theta3).*2.67415e-8+cos(theta1).*cos(theta3).*sin(theta2).*2.67415e-8)+(cos(theta2).*sin(theta1).*sin(theta3)+cos(theta3).*sin(theta1).*sin(theta2)).*(cos(theta1).*sin(theta2).*sin(theta3).*(-1.0425e-2)+cos(theta1).*cos(theta2).*cos(theta3).*1.0425e-2+cos(theta1).*cos(theta2).*sin(theta3).*2.67415e-8+cos(theta1).*cos(theta3).*sin(theta2).*2.67415e-8)+(sin(theta1).*sin(theta2).*sin(theta3)-cos(theta2).*cos(theta3).*sin(theta1)).*(cos(theta1).*sin(theta2).*sin(theta3).*(-2.67415e-8)+cos(theta1).*cos(theta2).*cos(theta3).*2.67415e-8+cos(theta1).*cos(theta2).*sin(theta3).*7.5434e-2+cos(theta1).*cos(theta3).*sin(theta2).*7.5434e-2)-(sin(theta1).*sin(theta2).*sin(theta3)-cos(theta2).*cos(theta3).*sin(theta1)).*(sin(theta1).*(-2.74946e-3)+cos(theta1).*sin(theta2).*sin(theta3).*2.67415e-8-cos(theta1).*cos(theta2).*cos(theta3).*2.67415e-8+cos(theta1).*cos(theta2).*sin(theta3).*1.0425e-2+cos(theta1).*cos(theta3).*sin(theta2).*1.0425e-2))-cos(theta1).*((sin(theta1).*sin(theta2).*sin(theta3)-cos(theta2).*cos(theta3).*sin(theta1)).*(cos(theta2).*sin(theta1).*sin(theta3).*7.5434e-2+cos(theta3).*sin(theta1).*sin(theta2).*7.5434e-2-sin(theta1).*sin(theta2).*sin(theta3).*2.67415e-8+cos(theta2).*cos(theta3).*sin(theta1).*2.67415e-8)-(sin(theta1).*sin(theta2).*sin(theta3)-cos(theta2).*cos(theta3).*sin(theta1)).*(cos(theta1).*2.74946e-3+cos(theta2).*sin(theta1).*sin(theta3).*1.0425e-2+cos(theta3).*sin(theta1).*sin(theta2).*1.0425e-2+sin(theta1).*sin(theta2).*sin(theta3).*2.67415e-8-cos(theta2).*cos(theta3).*sin(theta1).*2.67415e-8)+(cos(theta2).*sin(theta1).*sin(theta3)+cos(theta3).*sin(theta1).*sin(theta2)).*(cos(theta1).*2.13561e-9+cos(theta2).*sin(theta1).*sin(theta3).*2.67415e-8+cos(theta3).*sin(theta1).*sin(theta2).*2.67415e-8+sin(theta1).*sin(theta2).*sin(theta3).*7.5434e-2-cos(theta2).*cos(theta3).*sin(theta1).*7.5434e-2)+cos(theta1).*(cos(theta2).*sin(theta1).*sin(theta3).*2.13561e-9+cos(theta3).*sin(theta1).*sin(theta2).*2.13561e-9-sin(theta1).*sin(theta2).*sin(theta3).*2.74946e-3+cos(theta2).*cos(theta3).*sin(theta1).*2.74946e-3)+(cos(theta2).*sin(theta1).*sin(theta3)+cos(theta3).*sin(theta1).*sin(theta2)).*(cos(theta2).*sin(theta1).*sin(theta3).*2.67415e-8+cos(theta3).*sin(theta1).*sin(theta2).*2.67415e-8-sin(theta1).*sin(theta2).*sin(theta3).*1.0425e-2+cos(theta2).*cos(theta3).*sin(theta1).*1.0425e-2))))./2.0+((cos(theta2).*sin(theta1).*sin(theta3).*1.20975e-1+cos(theta3).*sin(theta1).*sin(theta2).*1.20975e-1).*(cos(theta2).*sin(theta1).*2.2140098-sin(theta1).*sin(theta2).*sin(theta3).*6.228833385e-1+cos(theta2).*cos(theta3).*sin(theta1).*6.228833385e-1))./2.0+((cos(theta2).*cos(theta3).*6.228833385e-1-sin(theta2).*sin(theta3).*6.228833385e-1).*(sin(theta2).*(4.3e+1./1.0e+2)+cos(theta2).*sin(theta3).*1.20975e-1+cos(theta3).*sin(theta2).*1.20975e-1))./2.0+(sin(theta1).*(sin(theta1).*((cos(theta1).*cos(theta2).*sin(theta3)+cos(theta1).*cos(theta3).*sin(theta2)).*(sin(theta1).*(-2.13561e-9)+cos(theta1).*sin(theta2).*sin(theta3).*7.5434e-2-cos(theta1).*cos(theta2).*cos(theta3).*7.5434e-2+cos(theta1).*cos(theta2).*sin(theta3).*2.67415e-8+cos(theta1).*cos(theta3).*sin(theta2).*2.67415e-8)+(cos(theta1).*cos(theta2).*sin(theta3)+cos(theta1).*cos(theta3).*sin(theta2)).*(cos(theta1).*sin(theta2).*sin(theta3).*(-1.0425e-2)+cos(theta1).*cos(theta2).*cos(theta3).*1.0425e-2+cos(theta1).*cos(theta2).*sin(theta3).*2.67415e-8+cos(theta1).*cos(theta3).*sin(theta2).*2.67415e-8)-sin(theta1).*(cos(theta1).*sin(theta2).*sin(theta3).*(-2.74946e-3)+cos(theta1).*cos(theta2).*cos(theta3).*2.74946e-3+cos(theta1).*cos(theta2).*sin(theta3).*2.13561e-9+cos(theta1).*cos(theta3).*sin(theta2).*2.13561e-9)+(cos(theta1).*sin(theta2).*sin(theta3)-cos(theta1).*cos(theta2).*cos(theta3)).*(cos(theta1).*sin(theta2).*sin(theta3).*(-2.67415e-8)+cos(theta1).*cos(theta2).*cos(theta3).*2.67415e-8+cos(theta1).*cos(theta2).*sin(theta3).*7.5434e-2+cos(theta1).*cos(theta3).*sin(theta2).*7.5434e-2)-(cos(theta1).*sin(theta2).*sin(theta3)-cos(theta1).*cos(theta2).*cos(theta3)).*(sin(theta1).*(-2.74946e-3)+cos(theta1).*sin(theta2).*sin(theta3).*2.67415e-8-cos(theta1).*cos(theta2).*cos(theta3).*2.67415e-8+cos(theta1).*cos(theta2).*sin(theta3).*1.0425e-2+cos(theta1).*cos(theta3).*sin(theta2).*1.0425e-2))-cos(theta1).*((cos(theta1).*cos(theta2).*sin(theta3)+cos(theta1).*cos(theta3).*sin(theta2)).*(cos(theta1).*2.13561e-9+cos(theta2).*sin(theta1).*sin(theta3).*2.67415e-8+cos(theta3).*sin(theta1).*sin(theta2).*2.67415e-8+sin(theta1).*sin(theta2).*sin(theta3).*7.5434e-2-cos(theta2).*cos(theta3).*sin(theta1).*7.5434e-2)+(cos(theta1).*cos(theta2).*sin(theta3)+cos(theta1).*cos(theta3).*sin(theta2)).*(cos(theta2).*sin(theta1).*sin(theta3).*2.67415e-8+cos(theta3).*sin(theta1).*sin(theta2).*2.67415e-8-sin(theta1).*sin(theta2).*sin(theta3).*1.0425e-2+cos(theta2).*cos(theta3).*sin(theta1).*1.0425e-2)-sin(theta1).*(cos(theta2).*sin(theta1).*sin(theta3).*2.13561e-9+cos(theta3).*sin(theta1).*sin(theta2).*2.13561e-9-sin(theta1).*sin(theta2).*sin(theta3).*2.74946e-3+cos(theta2).*cos(theta3).*sin(theta1).*2.74946e-3)+(cos(theta1).*sin(theta2).*sin(theta3)-cos(theta1).*cos(theta2).*cos(theta3)).*(cos(theta2).*sin(theta1).*sin(theta3).*7.5434e-2+cos(theta3).*sin(theta1).*sin(theta2).*7.5434e-2-sin(theta1).*sin(theta2).*sin(theta3).*2.67415e-8+cos(theta2).*cos(theta3).*sin(theta1).*2.67415e-8)-(cos(theta1).*sin(theta2).*sin(theta3)-cos(theta1).*cos(theta2).*cos(theta3)).*(cos(theta1).*2.74946e-3+cos(theta2).*sin(theta1).*sin(theta3).*1.0425e-2+cos(theta3).*sin(theta1).*sin(theta2).*1.0425e-2+sin(theta1).*sin(theta2).*sin(theta3).*2.67415e-8-cos(theta2).*cos(theta3).*sin(theta1).*2.67415e-8))))./2.0+(cos(theta1).*cos(theta2).*sin(theta3).*1.20975e-1+cos(theta1).*cos(theta3).*sin(theta2).*1.20975e-1).*(cos(theta1).*sin(theta2).*sin(theta3).*6.228833385e-1-cos(theta1).*cos(theta2).*cos(theta3).*6.228833385e-1))],[3,3]);
G_func = @(theta1,theta2,theta3)[0.0;sin(theta2).*(-3.877458010866e+1)-cos(theta2).*sin(theta3).*6.110485550685-cos(theta3).*sin(theta2).*6.110485550685;cos(theta2).*sin(theta3).*(-6.110485550685)-cos(theta3).*sin(theta2).*6.110485550685];

M = M_func(q(1), q(2), q(3));
C = C_func(q(1), q(2), q(3), q_dot(1), q_dot(2), q_dot(3));
G = G_func(q(1), q(2), q(3));


% coder.extrinsic('calculate_dynamics');
% [M,C,G] = calculate_dynamics(q,q_dot);

end
